simulink model "GFo_29bus"  (R2017a)
settings: Solver=ode1  StartTime=0.0  StopTime=4.5  FixedStep=Time_Step  RelTol=1e-3  EnableMultiTasking=on
PreLoadFcn:
  | Init_29bus;
InitFcn:
  | Init_29bus;
values from neighbouring files (symbols this model uses):
  Time_Step = 40e-6    (= 4e-05)    [Init_29bus.m]
  VSC01_Delta_P_Time_Step = 2    [Init_29bus.m]
  VSC01_Delta_P_Value = -0.2    [Init_29bus.m]
undefined symbols (not defined in the file or in its folder): D1, D11, Delta
libraries: powerlib x168, sps_avr x6, GFo_Lib x1
(part 2 of 5)

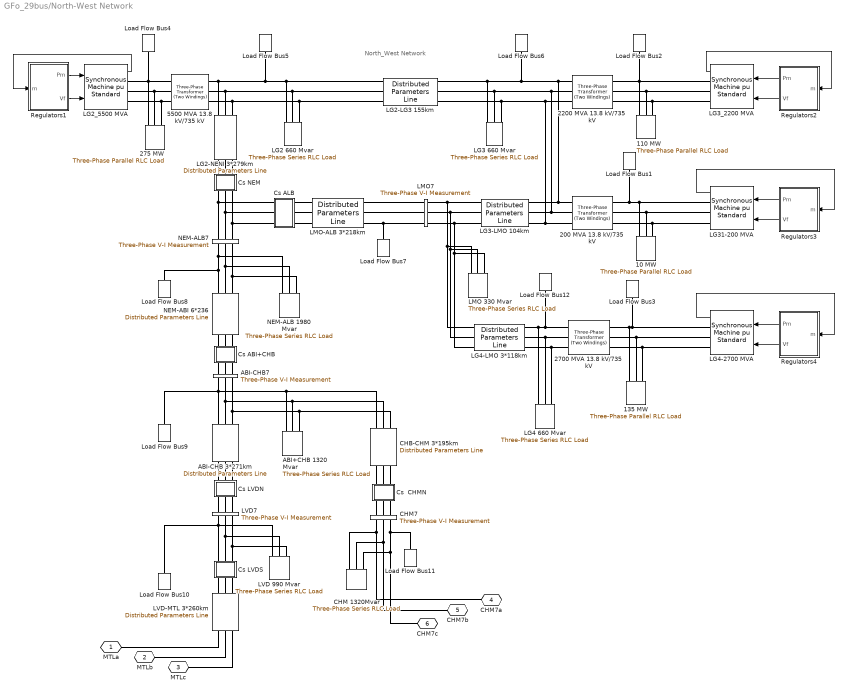
== system GFo_29bus/North-West Network ==
  note: North_West Network
  10 MW : powerlib/Elements/Three-Phase Parallel RLC Load  LConnTagsString=A|B|C  Configuration=Y (grounded)  NominalVoltage=(13800)*1  Vabc=[1e3 1e3 1e3]  Vabcp=[1e3 1e3 1e3]  NominalFrequency=60  UnbalancedPower=off  ActivePower=10000000  InductivePower=0  CapacitivePower=0  Pabc=[10e3 9e3 11e3]  QLabc=[100 90 110]  QCabc=[100 90 110]  Pabcp=[10e3 9e3 11e3]  QLabcp=[100 90 110]  QCabcp=[100 90 110]  Measurements=None  LoadType=constant PQ
  110 MW : powerlib/Elements/Three-Phase Parallel RLC Load  LConnTagsString=A|B|C  Configuration=Y (grounded)  NominalVoltage=(13800)*1  Vabc=[1e3 1e3 1e3]  Vabcp=[1e3 1e3 1e3]  NominalFrequency=60  UnbalancedPower=off  ActivePower=110000000  InductivePower=0  CapacitivePower=0  Pabc=[10e3 9e3 11e3]  QLabc=[100 90 110]  QCabc=[100 90 110]  Pabcp=[10e3 9e3 11e3]  QLabcp=[100 90 110]  QCabcp=[100 90 110]  Measurements=None  LoadType=constant PQ
  135 MW : powerlib/Elements/Three-Phase Parallel RLC Load  LConnTagsString=A|B|C  Configuration=Y (grounded)  NominalVoltage=(13800)*1  Vabc=[1e3 1e3 1e3]  Vabcp=[1e3 1e3 1e3]  NominalFrequency=60  UnbalancedPower=off  ActivePower=135000000  InductivePower=0  CapacitivePower=0  Pabc=[10e3 9e3 11e3]  QLabc=[100 90 110]  QCabc=[100 90 110]  Pabcp=[10e3 9e3 11e3]  QLabcp=[100 90 110]  QCabcp=[100 90 110]  Measurements=None  LoadType=constant PQ
  200 MVA 13.8 kV/735 kV : powerlib/Elements/Three-Phase Transformer (Two Windings)  Winding1Connection=Delta (D1)  Winding2Connection=Yg  CoreType=Three single-phase transformers  SetSaturation=off  Hysteresis=off  DataFile='basic_model'  SetInitialFlux=off  Measurements=None  UNITS=pu  NominalPower=[ 200e6 60 ]  Winding1="[ 13.8e3 0.002  0.0]"  Winding2=[ 735e3 0.002 0.12]  Rm=500  Lm=500  L0=0.5  Saturation="[ 0,0  ;  0.005,1.2  ;  1.0,1.4 ]"  InitialFluxes=[ 0.8 , -0.8 , 0.7 ]  MoreParameters=off  BreakLoop=off  DataType=off  TransfoNumber=0
  2200 MVA 13.8 kV/735 kV : powerlib/Elements/Three-Phase Transformer (Two Windings)  Winding1Connection=Delta (D1)  Winding2Connection=Yg  CoreType=Three single-phase transformers  SetSaturation=off  Hysteresis=off  DataFile='basic_model'  SetInitialFlux=off  Measurements=None  UNITS=pu  NominalPower=[ 2200e6 60 ]  Winding1="[ 13.8e3 0.002  0.0]"  Winding2=[ 735e3 0.002 0.12]  Rm=500  Lm=500  L0=0.5  Saturation="[ 0,0  ;  0.005,1.2  ;  1.0,1.4 ]"  InitialFluxes=[ 0.8 , -0.8 , 0.7 ]  MoreParameters=off  BreakLoop=off  DataType=off  TransfoNumber=0
  2700 MVA 13.8 kV/735 kV : powerlib/Elements/Three-Phase Transformer (Two Windings)  Winding1Connection=Delta (D1)  Winding2Connection=Yg  CoreType=Three single-phase transformers  SetSaturation=off  Hysteresis=off  DataFile='basic_model'  SetInitialFlux=off  Measurements=None  UNITS=pu  NominalPower=[ 2700e6 60 ]  Winding1="[ 13.8e3 0.002  0.0]"  Winding2=[ 735e3 0.002 0.12]  Rm=500  Lm=500  L0=0.5  Saturation="[ 0,0  ;  0.005,1.2  ;  1.0,1.4 ]"  InitialFluxes=[ 0.8 , -0.8 , 0.7 ]  MoreParameters=off  BreakLoop=off  DataType=off  TransfoNumber=0
  275 MW : powerlib/Elements/Three-Phase Parallel RLC Load  LConnTagsString=A|B|C  Configuration=Y (grounded)  NominalVoltage=(13800)*1  Vabc=[1e3 1e3 1e3]  Vabcp=[1e3 1e3 1e3]  NominalFrequency=60  UnbalancedPower=off  ActivePower=275000000  InductivePower=0  CapacitivePower=0  Pabc=[10e3 9e3 11e3]  QLabc=[100 90 110]  QCabc=[100 90 110]  Pabcp=[10e3 9e3 11e3]  QLabcp=[100 90 110]  QCabcp=[100 90 110]  Measurements=None  LoadType=constant PQ
  5500 MVA 13.8 kV/735 kV : powerlib/Elements/Three-Phase Transformer (Two Windings)  Winding1Connection=Delta (D1)  Winding2Connection=Yg  CoreType=Three single-phase transformers  SetSaturation=off  Hysteresis=off  DataFile='basic_model'  SetInitialFlux=off  Measurements=None  UNITS=pu  NominalPower=[ 5500e6 60 ]  Winding1="[ 13.8e3 0.002  0.0]"  Winding2=[ 735e3 0.002 0.12]  Rm=500  Lm=500  L0=0.5  Saturation="[ 0,0  ;  0.005,1.2  ;  1.0,1.4 ]"  InitialFluxes=[ 0.8 , -0.8 , 0.7 ]  MoreParameters=off  BreakLoop=off  DataType=off  TransfoNumber=0
  ABI+CHB 1320 Mvar : powerlib/Elements/Three-Phase Series RLC Load  LConnTagsString=A|B|C  Configuration=Y (grounded)  NominalVoltage=735e3  Vabc=[1e3 1e3 1e3]  Vabcp=[1e3 1e3 1e3]  NominalFrequency=60  UnbalancedPower=off  ActivePower=4400000  InductivePower=1320e6  CapacitivePower=0  Pabc=[10e3 9e3 11e3]  QLabc=[100 90 110]  QCabc=[100 90 110]  Pabcp=[10e3 9e3 11e3]  QLabcp=[100 90 110]  QCabcp=[100 90 110]  Measurements=None  LoadType=constant Z
  ABI-CHB 3*271km : powerlib/Elements/Distributed Parameters Line  Phases=3  Frequency=60  Resistance="[0.01273  0.3864]/3"  Inductance="[0.9337e-3  4.1264e-3]/3"  Capacitance=[12.74e-9 7.751e-9]*3  Length=271  x1=[-0.00156 9.5951452421556e-08 0 0;-0.00152 9.70899498769542e-08 0 0;-0.00148 9.82063699150184e-08 0 0;-0.00144 9.93004586714597e-08 0 0;-0.0014 1.0037196735993e-07 0 0;-0.00136 1.01420652328593e-07 0 0;-0.00132 1.02446275115531e-07 0 0;-0.00128 1.03448602502967e-07 0 0;-0.00124 1.04427406570297e-07 0 0;-0.0012 1.05382464745916e-07 0 0;-0.00116 1.06313559857832e-07 0 0;-0.00112 1.07220480183045e-07 0 0;-0.00108 1.08103019495694e-07 0 0;-0.00104 1.08960977113951e-07 0 0;-0.001 1.09794157945652e-07 0 0;-0.00096 1.1060237253266e-07 216619.58458071 -655246.59132654;-0.00092 1.11385437093949e-07 226475.422537365 -651905.728699672;-0.00088 1.12143173567389e-07 236279.761935975 -648416.628331894;-0.00084 1.12875409650242e-07 246030.373354311 -644780.083614539;-0.0008 1.13581978838336e-07 255725.039587421 -640996.921466518;-0.00076 1.14262720463932e-07 265361.556151809 -637068.002146277;-0.00072 1.14917479732254e-07 274937.731786708 -632994.219056188;-0.00068 1.15546107756691e-07 284451.38895236 -628776.498539396;-0.00064 1.16148461592652e-07 293900.36432517 -624415.799669173;-0.0006 1.16724404270068e-07 303282.50928962 -619913.114030838;-0.00056 1.17273804824541e-07 312595.690426855 -615269.465496275;-0.00052 1.17796538327124e-07 321837.789999797 -610485.909991117;-0.00048 1.18292485912725e-07 331006.706434705 -605563.535254633;-0.00044 1.1876153480714e-07 340100.354799049 -600503.460592389;-0.0004 1.19203578352696e-07 349116.667275612 -595306.836621728;-0.00036 1.19618516032503e-07 358053.593632691 -589974.845010127;-0.00032 1.20006253493309e-07 366909.101690301 -584508.698206496;-0.00028 1.20366702566962e-07 375681.177782275 -578909.639165482;-0.00024 1.20699781290449e-07 384367.827214159 -573178.941064826;-0.0002 1.21005413924541e-07 392967.074716781 -567317.907015856;-0.00016 1.21283530971012e-07 401476.964895416 -561327.869767173;-0.00012 1.21534069188446e-07 409895.562674423 -555210.191401589;-8e-05 1.21756971606611e-07 418220.953737267 -548966.26302641;-4e-05 1.21952187539421e-07 426451.244961816 -542597.504457102]  x2=[-0.00156 2.08994673487687e-07 0 0;-0.00152 2.11355075811643e-07 0 0;-0.00148 2.13667417814008e-07 0 0;-0.00144 2.15931173688151e-07 0 0;-0.0014 2.18145828675509e-07 0 0;-0.00136 2.20310879182635e-07 0 0;-0.00132 2.22425832895715e-07 0 0;-0.00128 2.24490208892514e-07 0 0;-0.00124 2.26503537751732e-07 0 0;-0.0012 2.28465361659748e-07 0 0;-0.00116 2.30375234514724e-07 0 0;-0.00112 2.32232722028042e-07 0 0;-0.00108 2.34037401823062e-07 0 0;-0.00104 2.35788863531159e-07 0 0;-0.001 2.37486708885046e-07 0 0;-0.00096 2.39130551809331e-07 -50306.9183180223 -677474.462196763;-0.00092 2.40720018508308e-07 -40085.5444534979 -678156.068059365;-0.00088 2.42254747550957e-07 -29855.0554818478 -678683.467080259;-0.00084 2.4373438995313e-07 -19617.7777280401 -679056.539333457;-0.0008 2.45158609256902e-07 -9376.03906075358 -679275.199985543;-0.00076 2.46527081607088e-07 867.831636959905 -679339.399314973;-0.00072 2.47839495824875e-07 11111.5049972429 -679249.122723373;-0.00068 2.49095553478589e-07 21352.6516971111 -679004.390738859;-0.00064 2.5029496895155e-07 31588.9429881209 -678605.259011377;-0.0006 2.51437469507023e-07 41818.0512259065 -678051.818300037;-0.00056 2.52522795350234e-07 52037.6503994669 -677344.194452486;-0.00052 2.53550699687447e-07 62245.4166600801 -676482.548376285;-0.00048 2.5452094878208e-07 72439.0288497263 -675467.076002319;-0.00044 2.55433322007854e-07 82616.1690288997 -674298.00824025;-0.0004 2.56287611898967e-07 92774.5230036874 -672975.610926006;-0.00036 2.57083624197264e-07 102911.780851998 -671500.184761332;-0.00032 2.57821177896413e-07 113025.637448815 -669872.065245414;-0.00028 2.58500105283064e-07 123113.792990369 -668091.62259859;-0.00024 2.59120251974984e-07 133173.953517084 -666159.261678164;-0.0002 2.59681476956162e-07 143203.831435213 -664075.421886345;-0.00016 2.60183652608878e-07 153201.146037011 -661840.577070332;-0.00012 2.6062666474272e-07 163163.624019351 -659455.235414563;-8e-05 2.61010412620547e-07 173089.000000652 -656919.93932516;-4e-05 2.61334808981402e-07 182975.017036008 -654235.265306591]  x3=[-0.00156 -1.04791549679137e-10 0 0;-0.00152 -8.57007981393384e-11 0 0;-0.00148 -6.65905589770951e-11 0 0;-0.00144 -4.74651776959928e-11 0 0;-0.0014 -2.83290032428046e-11 0 0;-0.00136 -9.18638701857813e-12 0 0;-0.00132 9.95831811083642e-12 0 0;-0.00128 2.91007588045895e-11 0 0;-0.00124 4.82365822367446e-11 0 0;-0.0012 6.73614370860738e-11 0 0;-0.00116 8.64709745255098e-11 0 0;-0.00112 1.05560849211033e-10 0 0;-0.00108 1.24626720269763e-10 0 0;-0.00104 1.43664252287039e-10 0 0;-0.001 1.62669116292252e-10 0 0;-0.00096 1.8163699074322e-10 85.0496761443598 864.700572722881;-0.00092 2.00563562508863e-10 72.0004876131748 865.884385233979;-0.00088 2.19444527849978e-10 58.9349267920121 866.871303102944;-0.00084 2.38275593397869e-10 45.8559646767302 867.661101913164;-0.0008 2.57052477130623e-10 32.7665753105259 868.253602071198;-0.00076 2.75770909346803e-10 19.6697351076627 868.648668847622;-0.00072 2.94426633636345e-10 6.56842217666069 868.846212407657;-0.00068 3.13015407848425e-10 -6.53438435690062 868.846187831601;-0.00064 3.3153300505609e-10 -19.6357050278094 868.648595125043;-0.0006 3.49975214517425e-10 -32.7325607087259 868.25347921886;-0.00056 3.68337842633035e-10 -45.8219732876108 867.660929959001;-0.00052 3.86616713899642e-10 -58.9009663449219 866.871082086059;-0.00048 4.04807671859548e-10 -71.9665658304266 865.884115204629;-0.00044 4.22906580045786e-10 -85.0158007394746 864.700253742467;-0.0004 4.40909322922712e-10 -98.0457037885795 863.319766899462;-0.00036 4.58811806821846e-10 -111.053312090153 861.742968586416;-0.00032 4.76609960872733e-10 -124.03566782624 859.970217353669;-0.00028 4.94299737928627e-10 -136.989818921102 858.001916309563;-0.00024 5.11877115486776e-10 -149.912819712491 855.838513028782;-0.0002 5.29338096603103e-10 -162.80173162147 853.480499450574;-0.00016 5.46678710801079e-10 -175.653623820621 850.928411766894;-0.00012 5.63895014974577e-10 -188.465573900487 848.182830300473;-8e-05 5.80983094284492e-10 -201.234668534106 845.244379372858;-4e-05 5.97939063048952e-10 -213.958004139475 842.113727162451]  x4=[-0.00156 9.60954535339062e-10 0 0;-0.00152 9.59976323627074e-10 0 0;-0.00148 9.58779821577575e-10 0 0;-0.00144 9.57365301264816e-10 0 0;-0.0014 9.55733084338515e-10 0 0;-0.00136 9.53883541950726e-10 0 0;-0.00132 9.5181709467144e-10 0 0;-0.00128 9.49534212392946e-10 0 0;-0.00124 9.47035414222988e-10 0 0;-0.0012 9.44321268366722e-10 0 0;-0.00116 9.41392391997508e-10 0 0;-0.00112 9.38249451116577e-10 0 0;-0.00108 9.34893160401581e-10 0 0;-0.00104 9.31324283044084e-10 0 0;-0.001 9.27543630576022e-10 0 0;-0.00096 9.23552062685162e-10 -872.254416614129 -15817.4970067936;-0.00092 9.19350487019622e-10 -633.642051346427 -15828.8524142298;-0.00088 9.14939858981474e-10 -394.885601340545 -15836.6084771291;-0.00084 9.10321181509499e-10 -156.039357754267 -15840.7634318299;-0.0008 9.05495504851124e-10 82.8423678363377 -15841.3163335312;-0.00076 9.00463926323607e-10 321.7052557869 -15838.2670565079;-0.00072 8.95227590064514e-10 560.494990736563 -15831.6162941394;-0.00068 8.89787686771555e-10 799.157273958836 -15821.3655587517;-0.00064 8.84145453431825e-10 1037.63783570865 -15807.5171812735;-0.0006 8.78302173040531e-10 1275.88244756283 -15790.0743107065;-0.00056 8.72259174309243e-10 1513.83693475118 -15769.0409134091;-0.00052 8.6601783136376e-10 1751.44718847534 -15744.4217721944;-0.00048 8.59579563431644e-10 1988.65917821267 -15716.2224852428;-0.00044 8.52945834519503e-10 2225.41896400235 -15684.449464829;-0.0004 8.46118153080083e-10 2461.67270871081 -15649.1099358638;-0.00036 8.39098071669265e-10 2697.36669027387 -15610.2119342514;-0.00032 8.31887186593023e-10 2932.44731391266 -15567.7643050618;-0.00028 8.24487137544439e-10 3166.86112432061 -15521.77670052;-0.00024 8.16899607230852e-10 3400.55481781874 -15472.2595778106;-0.0002 8.09126320991223e-10 3633.47525447644 -15419.2241967002;-0.00016 8.01169046403809e-10 3865.56947019502 -15362.6826169773;-0.00012 7.9302959288423e-10 4096.78468875133 -15302.6476957094;-8e-05 7.84709811274025e-10 4327.06833379859 -15239.1330843199;-4e-05 7.76211593419786e-10 4556.36804082179 -15172.1532254837]  x5=0.00153261764655846  V1=ones(3,3)  V2=ones(3,3)  I1=ones(3,3)  I2=ones(3,3)  nHarmo=1  Measurements=None
      settings: AttributesFormatString=\n  SourceProductName=Simscape Power Systems
  ABI-CHB7 : powerlib/Measurements/Three-Phase V-I Measurement  VoltageMeasurement=no  SetLabelV=on  LabelV=Vabc_ABI7  Vpu=on  VpuLL=off  CurrentMeasurement=no  SetLabelI=off  LabelI=A1  Ipu=off  Pbase=100e6  Vbase=500e3  OutputType=Magnitude  PhasorSimulation=off  PSBequivalent=0
  CHB-CHM 3*195km : powerlib/Elements/Distributed Parameters Line  Phases=3  Frequency=60  Resistance="[0.01273  0.3864]/3"  Inductance="[0.9337e-3  4.1264e-3]/3"  Capacitance=[12.74e-9 7.751e-9]*3  Length=195  x1=[-0.00112 1.07244333430672e-07 0 0;-0.00108 1.08126069397218e-07 0 0;-0.00104 1.08983218428023e-07 0 0;-0.001 1.09815585614788e-07 0 0;-0.00096 1.10622981684394e-07 0 0;-0.00092 1.11405223041937e-07 0 0;-0.00088 1.12162131812478e-07 0 0;-0.00084 1.12893535881489e-07 0 0;-0.0008 1.13599268933994e-07 0 0;-0.00076 1.14279170492381e-07 0 0;-0.00072 1.149330859529e-07 0 0;-0.00068 1.15560866620814e-07 284451.38895236 -628776.498539396;-0.00064 1.16162369744213e-07 293900.36432517 -624415.799669173;-0.0006 1.16737458546474e-07 303282.50928962 -619913.114030838;-0.00056 1.17286002257362e-07 312595.690426855 -615269.465496275;-0.00052 1.17807876142768e-07 321837.789999797 -610485.909991117;-0.00048 1.18302961533072e-07 331006.706434705 -605563.535254633;-0.00044 1.18771145850124e-07 340100.354799049 -600503.460592389;-0.0004 1.19212322632848e-07 349116.667275612 -595306.836621728;-0.00036 1.19626391561449e-07 358053.593632691 -589974.845010127;-0.00032 1.20013258480223e-07 366909.101690301 -584508.698206496;-0.00028 1.20372835418969e-07 375681.177782275 -578909.639165482;-0.00024 1.20705040612991e-07 384367.827214159 -573178.941064826;-0.0002 1.21009798521694e-07 392967.074716781 -567317.907015856;-0.00016 1.21287039845758e-07 401476.964895416 -561327.869767173;-0.00012 1.21536701542895e-07 409895.562674423 -555210.191401589;-8e-05 1.2175872684219e-07 418220.953737267 -548966.26302641;-4e-05 1.21953065257003e-07 426451.244961816 -542597.504457102]  x2=[-0.00112 7.55642474220007e-08 0 0;-0.00108 7.61098867769976e-08 0 0;-0.00104 7.6638219400085e-08 0 0;-0.001 7.71491251529807e-08 0 0;-0.00096 7.76424878601224e-08 0 0;-0.00092 7.8118195335085e-08 0 0;-0.00088 7.8576139406091e-08 0 0;-0.00084 7.90162159406078e-08 0 0;-0.0008 7.94383248690265e-08 0 0;-0.00076 7.9842370207417e-08 0 0;-0.00072 8.02282600793536e-08 0 0;-0.00068 8.05959067368072e-08 200726.403510761 -641022.029740575;-0.00064 8.09452265800983e-08 210369.549035787 -637922.423631795;-0.0006 8.1276140176907e-08 219964.858339513 -634677.75946509;-0.00056 8.15885722803351e-08 229510.149531348 -631288.775049111;-0.00052 8.18824518460165e-08 239003.25209439 -627756.241009687;-0.00048 8.21577120482723e-08 248442.007378983 -624080.960614598;-0.00044 8.24142902953063e-08 257824.26909357 -620263.76959091;-0.0004 8.26521282434376e-08 267147.903792748 -616305.535934943;-0.00036 8.28711718103681e-08 276410.791362388 -612207.159714898;-0.00032 8.30713711874794e-08 285610.825501738 -607969.572866183;-0.00028 8.32526808511596e-08 294745.914202371 -603593.738979505;-0.00024 8.34150595731549e-08 303813.980223895 -599080.653081753;-0.0002 8.3558470429944e-08 312812.961566297 -594431.341409743;-0.00016 8.3682880811135e-08 321740.811938822 -589646.861176853;-0.00012 8.37882624268799e-08 330595.501225287 -584728.300332629;-8e-05 8.38745913143081e-08 339375.015945708 -579676.777315392;-4e-05 8.39418478429752e-08 348077.359714148 -574493.440797913]  x3=[-0.00112 4.95882150276911e-10 0 0;-0.00108 4.95457745542146e-10 0 0;-0.00104 4.9492067798869e-10 0 0;-0.001 4.94271069741073e-10 0 0;-0.00096 4.9350906851461e-10 0 0;-0.00092 4.92634847581807e-10 0 0;-0.00088 4.91648605732966e-10 0 0;-0.00084 4.90550567230979e-10 0 0;-0.0008 4.89340981760331e-10 0 0;-0.00076 4.88020124370327e-10 0 0;-0.00072 4.86588295412549e-10 0 0;-0.00068 4.85045820472552e-10 1577.42073477442 -3661.80221392756;-0.00064 4.83393050295836e-10 1632.45704438713 -3637.60049775401;-0.0006 4.81630360708088e-10 1687.12214734566 -3612.57162259661;-0.00056 4.79758152529718e-10 1741.403613277 -3586.72127980571;-0.00052 4.7777685148472e-10 1795.28909904391 -3560.05534752636;-0.00048 4.75686908103867e-10 1848.76635155161 -3532.57988936159;-0.00044 4.73488797622261e-10 1901.82321053405 -3504.30115299364;-0.0004 4.71183019871269e-10 1954.44761131904 -3475.22556876332;-0.00036 4.68770099164867e-10 2006.62758757165 -3445.35974820772;-0.00032 4.66250584180416e-10 2058.35127401527 -3414.7104825569;-0.00028 4.63625047833897e-10 2109.60690912964 -3383.28474118956;-0.00024 4.60894087149632e-10 2160.38283782535 -3351.08967004827;-0.0002 4.58058323124531e-10 2210.66751409409 -3318.13259001459;-0.00016 4.55118400586877e-10 2260.44950363411 -3284.42099524429;-0.00012 4.52074988049705e-10 2309.71748645029 -3249.96255146331;-8e-05 4.48928777558778e-10 2358.4602594282 -3214.76509422461;-4e-05 4.45680484535232e-10 2406.66673888162 -3178.83662712644]  x4=[-0.00112 1.21600407393123e-10 0 0;-0.00108 1.29687420233768e-10 0 0;-0.00104 1.3774494327343e-10 0 0;-0.001 1.45771144300853e-10 0 0;-0.00096 1.53764198227138e-10 0 0;-0.00092 1.61722287500753e-10 0 0;-0.00088 1.69643602520824e-10 0 0;-0.00084 1.77526342048625e-10 0 0;-0.0008 1.85368713617167e-10 0 0;-0.00076 1.93168933938784e-10 0 0;-0.00072 2.00925229310641e-10 0 0;-0.00068 2.08635836018058e-10 1976.82314553332 -10994.7955965049;-0.00064 2.16299000735563e-10 2142.38966517679 -10963.7374282637;-0.0006 2.23912980925585e-10 2307.46902388557 -10930.1862006786;-0.00056 2.31476045234687e-10 2472.0236840371 -10894.1495430093;-0.00052 2.38986473887267e-10 2636.01622732069 -10855.6356496811;-0.00048 2.46442559076617e-10 2799.40936324623 -10814.6532784211;-0.00044 2.53842605353263e-10 2962.16593762364 -10771.2117482673;-0.0004 2.61184930010497e-10 3124.24894101147 -10725.3209374489;-0.00036 2.6846786346701e-10 3285.62151713249 -10676.9912811405;-0.00032 2.75689749646538e-10 3446.2469712545 -10626.2337690892;-0.00028 2.82848946354444e-10 3606.08877853442 -10573.0599431156;-0.00024 2.89943825651134e-10 3765.11059232369 -10517.4818944891;-0.0002 2.96972774222241e-10 3923.2762524332 -10459.5122611787;-0.00016 3.03934193745473e-10 4080.54979335579 -10399.1642249791;-0.00012 3.10826501254065e-10 4236.89545244454 -10336.4515085133;-8e-05 3.17648129496725e-10 4392.27767804483 -10271.3883721123;-4e-05 3.24397527294018e-10 4546.66113757852 -10203.9896105721]  x5=0.0011028060556417  V1=ones(3,3)  V2=ones(3,3)  I1=ones(3,3)  I2=ones(3,3)  nHarmo=1  Measurements=None
      settings: AttributesFormatString=\n  SourceProductName=Simscape Power Systems
  CHM 1320Mvar : powerlib/Elements/Three-Phase Series RLC Load  LConnTagsString=A|B|C  Configuration=Y (grounded)  NominalVoltage=735e3  Vabc=[1e3 1e3 1e3]  Vabcp=[1e3 1e3 1e3]  NominalFrequency=60  UnbalancedPower=off  ActivePower=4400000  InductivePower=1320e6  CapacitivePower=0  Pabc=[10e3 9e3 11e3]  QLabc=[100 90 110]  QCabc=[100 90 110]  Pabcp=[10e3 9e3 11e3]  QLabcp=[100 90 110]  QCabcp=[100 90 110]  Measurements=None  LoadType=constant Z
  CHM7 : powerlib/Measurements/Three-Phase V-I Measurement  VoltageMeasurement=no  SetLabelV=on  LabelV=Vabc_CHM7  Vpu=on  VpuLL=off  CurrentMeasurement=no  SetLabelI=off  LabelI=A1  Ipu=off  Pbase=100e6  Vbase=735e3  OutputType=Magnitude  PhasorSimulation=off  PSBequivalent=0
  "Cs  CHMN " : Subsystem  mask{Xc=25/3}
      mask prompts: Xc "Condensator Reactance at  60Hz  (ohm):"
      mask help: Series Compensation
      mask init:
      | Cs=1/Xc/(2*pi*60);
      mask Display: disp('Cs')
  "Cs ABI+CHB " : Subsystem  mask{Xc=25/6}
      mask prompts: Xc "Condensator Reactance at  60Hz  (ohm):"
      mask help: Series Compensation
      mask init:
      | Cs=1/Xc/(2*pi*60);
      mask Display: disp('Cs')
  Cs ALB : Subsystem  mask{Xc=16/3}
      mask prompts: Xc "Reactance @ 60Hz du condensateur (ohm):"
      mask init:
      | Cs=1/Xc/(2*pi*60);
      mask Display: disp('Cs')
  "Cs LVDN " : Subsystem  mask{Xc=34/3}
      mask prompts: Xc "Condensator Reactance at  60Hz  (ohm):"
      mask help: Series Compensation
      mask init:
      | Cs=1/Xc/(2*pi*60);
      mask Display: disp('Cs')
  "Cs LVDS " : Subsystem  mask{Xc=34/3}
      mask prompts: Xc "Condensator Reactance at  60Hz  (ohm):"
      mask help: Series Compensation
      mask init:
      | Cs=1/Xc/(2*pi*60);
      mask Display: disp('Cs')
  "Cs NEM " : Subsystem  mask{Xc=16/3}
      mask prompts: Xc "Condensator Reactance at  60Hz  (ohm):"
      mask help: Series Compensation
      mask init:
      | Cs=1/Xc/(2*pi*60);
      mask Display: disp('Cs')
  LG2 660 Mvar : powerlib/Elements/Three-Phase Series RLC Load  LConnTagsString=A|B|C  Configuration=Y (grounded)  NominalVoltage=735e3  Vabc=[1e3 1e3 1e3]  Vabcp=[1e3 1e3 1e3]  NominalFrequency=60  UnbalancedPower=off  ActivePower=2200000  InductivePower=660e6  CapacitivePower=0  Pabc=[10e3 9e3 11e3]  QLabc=[100 90 110]  QCabc=[100 90 110]  Pabcp=[10e3 9e3 11e3]  QLabcp=[100 90 110]  QCabcp=[100 90 110]  Measurements=None  LoadType=constant Z
  LG2-LG3 155km : powerlib/Elements/Distributed Parameters Line  Phases=3  Frequency=60  Resistance="[0.01273  0.3864]"  Inductance="[0.9337e-3  4.1264e-3]"  Capacitance=[12.74e-9 7.751e-9]  Length=155  x1=[-0.00088 4.73235624331992e-09 492216.116306252 -498778.900482482;-0.00084 4.72947863230192e-09 499681.229064062 -491300.088111067;-0.0008 4.72552557862823e-09 507032.71861945 -483709.558336407;-0.00076 4.72049798118915e-09 514268.913307088 -476009.037179515;-0.00072 4.71439698321699e-09 521388.167678706 -468200.275672495;-0.00068 4.70722397202608e-09 528388.862877254 -460285.049460374;-0.00064 4.69898057869729e-09 535269.407005016 -452265.158397336;-0.0006 4.6896686777072e-09 542028.235485591 -444142.426137446;-0.00056 4.67929038650177e-09 548663.811419669 -435918.699719975;-0.00052 4.66784806501494e-09 555174.625934506 -427595.849149389;-0.00048 4.65534431513192e-09 561559.198527027 -419175.766970137;-0.00044 4.64178198009763e-09 567816.077400483 -410660.367836293;-0.0004 4.62716414387009e-09 573943.839794576 -402051.588076187;-0.00036 4.61149413041919e-09 579941.09230898 -393351.385252099;-0.00032 4.59477550297087e-09 585806.471220193 -384561.737715121;-0.00028 4.57701206319682e-09 591538.642791629 -375684.644155307;-0.00024 4.55820785035008e-09 597136.303576907 -366722.123147178;-0.0002 4.53836714034648e-09 602598.180716236 -357676.212690722;-0.00016 4.51749444479238e-09 607923.032225855 -348548.969747969;-0.00012 4.49559450995874e-09 613109.647280451 -339342.469775253;-8e-05 4.47267231570189e-09 618156.846488488 -330058.806251276;-4e-05 4.44873307433114e-09 623063.48216039 -320700.090201062]  x2=[-0.00088 -1.8594565706245e-09 498841.55452554 -488122.876382841;-0.00084 -1.90046755388394e-09 506145.233646554 -480545.374264078;-0.0008 -1.94104638721055e-09 513333.819706248 -472858.600271255;-0.00076 -1.98118384332758e-09 520405.678082143 -465064.302310489;-0.00072 -2.02087079532365e-09 527359.200694629 -457164.252737921;-0.00068 -2.0600982187281e-09 534192.80637263 -449160.247956698;-0.00064 -2.09885719356314e-09 540904.941213144 -441054.108008481;-0.0006 -2.13713890637215e-09 547494.078934592 -432847.676159593;-0.00056 -2.17493465222374e-09 553958.721223878 -424542.818481865;-0.00052 -2.21223583669126e-09 560297.398077094 -416141.423428316;-0.00048 -2.24903397780702e-09 566508.668133786 -407645.401403729;-0.00044 -2.28532070799107e-09 572591.119004707 -399056.684330248;-0.0004 -2.32108777595389e-09 578543.367592983 -390377.225208069;-0.00036 -2.35632704857267e-09 584364.060408613 -381608.997671347;-0.00032 -2.3910305127407e-09 590051.873876247 -372753.99553941;-0.00028 -2.4251902771895e-09 595605.514636152 -363814.232363381;-0.00024 -2.45879857428322e-09 601023.719838313 -354791.740968313;-0.0002 -2.49184776178493e-09 606305.25742959 -345688.572990943;-0.00016 -2.52433032459438e-09 611448.926433881 -336506.798413165;-0.00012 -2.55623887645692e-09 616453.557225212 -327248.50509134;-8e-05 -2.58756616164302e-09 621318.011793699 -317915.798281528;-4e-05 -2.61830505659818e-09 626041.184004323 -308510.800160775]  x3=[-0.00088 9.57977380688901e-12 1822.65778344413 -2130.15037170099;-0.00084 9.18431506304634e-12 1854.57117293959 -2102.42438377255;-0.0008 8.78676788516048e-12 1886.06284894347 -2074.22032266978;-0.00076 8.3872226720314e-12 1917.1256505202 -2045.54460175295;-0.00072 7.98577027679503e-12 1947.7525142566 -2016.40374163371;-0.00068 7.58250198626407e-12 1977.93647586796 -1986.80436869234;-0.00064 7.17750950017013e-12 2007.6706717817 -1956.75321357101;-0.0006 6.77088491031207e-12 2036.94834069809 -1926.25710964323;-0.00056 6.36272067961503e-12 2065.76282512771 -1895.32299146005;-0.00052 5.95310962110521e-12 2094.10757290527 -1863.95789317318;-0.00048 5.54214487680498e-12 2121.97613867956 -1832.16894693549;-0.00044 5.12991989655318e-12 2149.36218537906 -1799.96338127922;-0.0004 4.71652841675546e-12 2176.25948565292 -1767.34851947228;-0.00036 4.30206443906937e-12 2202.661923287 -1734.33177785297;-0.00032 3.88662220902926e-12 2228.56349459468 -1700.92066414361;-0.00028 3.47029619461563e-12 2253.95830978199 -1667.12277574334;-0.00024 3.05318106477389e-12 2278.84059428697 -1632.94579800053;-0.0002 2.63537166788754e-12 2303.2046900927 -1598.39750246517;-0.00016 2.21696301021039e-12 2327.04505701389 -1563.48574512175;-0.00012 1.79805023426299e-12 2350.35627395669 -1528.21846460281;-8e-05 1.37872859719805e-12 2373.13304015141 -1492.60368038382;-4e-05 9.59093449139748e-13 2395.37017635782 -1456.64949095957]  x4=[-0.00088 -6.8062295315058e-12 1450.90460658014 -1864.19450277471;-0.00084 -6.45732020575493e-12 1478.84974910908 -1842.10455115884;-0.0008 -6.10694254107482e-12 1506.45861395813 -1819.59572085367;-0.00076 -5.7551762103249e-12 1533.72492310951 -1796.6731301731;-0.00072 -5.40210120213528e-12 1560.64247643966 -1773.34199151658;-0.00068 -5.04779780271803e-12 1587.20515312907 -1749.60761018384;-0.00064 -4.6923465776108e-12 1613.40691305413 -1725.47538316852;-0.0006 -4.33582835335689e-12 1639.2417981606 -1700.95079793093;-0.00056 -3.97832419912602e-12 1664.70393381838 -1676.03943115027;-0.00052 -3.61991540827988e-12 1689.7875301574 -1650.74694745651;-0.00048 -3.26068347988671e-12 1714.48688338418 -1625.07909814234;-0.00044 -2.90071010018915e-12 1738.79637707878 -1599.04171985533;-0.0004 -2.54007712402947e-12 1762.71048347197 -1572.64073327078;-0.00036 -2.17886655623648e-12 1786.22376470219 -1545.88214174535;-0.00032 -1.81716053297834e-12 1809.33087405206 -1518.77202995202;-0.00028 -1.45504130308553e-12 1832.02655716417 -1491.3165624964;-0.00024 -1.09259120934814e-12 1854.3056532359 -1463.52198251504;-0.0002 -7.29892669791852e-13 1876.16309619294 -1435.39461025573;-0.00016 -3.67028158936777e-13 1897.59391584125 -1406.94084164037;-0.00012 -4.08018904347539e-15 1918.59323899724 -1378.16714681056;-8e-05 3.58868708649629e-13 1939.15629059594 -1349.08006865637;-4e-05 7.21736002693137e-13 1959.27839477672 -1319.68622132853]  x5=0.000876589428843401  V1=ones(3,3)  V2=ones(3,3)  I1=ones(3,3)  I2=ones(3,3)  nHarmo=1  Measurements=None
      settings: AttributesFormatString=\n  SourceProductName=Simscape Power Systems
  LG2-NENI 3*279km : powerlib/Elements/Distributed Parameters Line  Phases=3  Frequency=60  Resistance="[0.01273  0.3864]/3"  Inductance="[0.9337e-3  4.1264e-3]/3"  Capacitance=[12.74e-9 7.751e-9]*3  Length=279  x1=[-0.0016 4.6006914312274e-09 0 0;-0.00156 4.61704685698524e-09 0 0;-0.00152 4.63235240610353e-09 0 0;-0.00148 4.64660459823237e-09 0 0;-0.00144 4.65980019254618e-09 0 0;-0.0014 4.67193618848062e-09 0 0;-0.00136 4.68300982641485e-09 0 0;-0.00132 4.69301858829912e-09 0 0;-0.00128 4.70196019822727e-09 0 0;-0.00124 4.70983262295433e-09 0 0;-0.0012 4.71663407235879e-09 0 0;-0.00116 4.72236299984972e-09 0 0;-0.00112 4.72701810271841e-09 0 0;-0.00108 4.73059832243461e-09 0 0;-0.00104 4.73310284488722e-09 0 0;-0.001 4.73453110056945e-09 469156.140703849 -520528.156335111;-0.00096 4.73488276470827e-09 476951.836643365 -513394.596336102;-0.00092 4.73415775733829e-09 484639.077848285 -506144.294833213;-0.00088 4.73235624331992e-09 492216.116306252 -498778.900482482;-0.00084 4.72947863230192e-09 499681.229064062 -491300.088111067;-0.0008 4.72552557862823e-09 507032.71861945 -483709.558336407;-0.00076 4.72049798118915e-09 514268.913307088 -476009.037179515;-0.00072 4.71439698321699e-09 521388.167678706 -468200.275672495;-0.00068 4.70722397202608e-09 528388.862877254 -460285.049460374;-0.00064 4.69898057869729e-09 535269.407005016 -452265.158397336;-0.0006 4.6896686777072e-09 542028.235485591 -444142.426137446;-0.00056 4.67929038650177e-09 548663.811419669 -435918.699719975;-0.00052 4.66784806501494e-09 555174.625934506 -427595.849149389;-0.00048 4.65534431513192e-09 561559.198527027 -419175.766970137;-0.00044 4.64178198009763e-09 567816.077400483 -410660.367836293;-0.0004 4.62716414387009e-09 573943.839794576 -402051.588076187;-0.00036 4.61149413041919e-09 579941.09230898 -393351.385252099;-0.00032 4.59477550297087e-09 585806.471220193 -384561.737715121;-0.00028 4.57701206319682e-09 591538.642791629 -375684.644155307;-0.00024 4.55820785035008e-09 597136.303576907 -366722.123147178;-0.0002 4.53836714034648e-09 602598.180716236 -357676.212690722;-0.00016 4.51749444479238e-09 607923.032225855 -348548.969747969;-0.00012 4.49559450995874e-09 613109.647280451 -339342.469775253;-8e-05 4.47267231570189e-09 618156.846488488 -330058.806251276;-4e-05 4.44873307433114e-09 623063.48216039 -320700.090201062]  x2=[-0.0016 5.75368748310283e-08 0 0;-0.00156 5.81983011827248e-08 0 0;-0.00152 5.88464937426131e-08 0 0;-0.00148 5.94813051172949e-08 0 0;-0.00144 6.0102590956138e-08 0 0;-0.0014 6.07102099841003e-08 0 0;-0.00136 6.13040240338548e-08 0 0;-0.00132 6.18838980772074e-08 0 0;-0.00128 6.24497002558012e-08 0 0;-0.00124 6.30013019111002e-08 0 0;-0.0012 6.35385776136446e-08 0 0;-0.00116 6.40614051915731e-08 0 0;-0.00112 6.4569665758403e-08 0 0;-0.00108 6.50632437400645e-08 0 0;-0.00104 6.55420269011811e-08 0 0;-0.001 6.60059063705907e-08 282256.24346152 -628817.283710635;-0.00096 6.64547766661023e-08 291706.090402666 -624489.689782335;-0.00092 6.68885357184817e-08 301089.60589442 -620020.092283949;-0.00088 6.73070848946608e-08 310404.65620628 -615409.507563403;-0.00084 6.77103290201665e-08 319649.123176135 -610658.984027902;-0.0008 6.80981764007619e-08 328820.904691916 -605769.601905532;-0.00076 6.84705388432976e-08 337917.915169601 -600742.472999624;-0.00072 6.8827331675765e-08 346938.086027456 -595578.740435938;-0.00068 6.9168473766551e-08 355879.366156415 -590279.578402729;-0.00064 6.9493887542886e-08 364739.722386483 -584846.191883746;-0.0006 6.98034990084834e-08 373517.139949062 -579279.816384227;-0.00056 7.00972377603662e-08 382209.622935091 -573581.717649958;-0.00052 7.0375037004875e-08 390815.1947489 -567753.191379454;-0.00048 7.06368335728574e-08 399331.89855767 -561795.562929326;-0.00044 7.08825679340314e-08 407757.797736399 -555710.187012905;-0.0004 7.11121842105225e-08 416090.976308277 -549498.447392199;-0.00036 7.13256301895694e-08 424329.539380358 -543161.756563228;-0.00032 7.15228573353973e-08 432471.613574446 -536701.555434843;-0.00028 7.1703820800254e-08 440515.347453083 -530119.313001069;-0.00024 7.18684794346081e-08 448458.911940553 -523416.526007072;-0.0002 7.20167957965061e-08 456300.500738791 -516594.718608813;-0.00016 7.21487361600864e-08 464038.33073813 -509655.442026466;-0.00012 7.22642705232481e-08 471670.642422755 -502600.274191683;-8e-05 7.23633726144734e-08 479195.700270808 -495430.81938879;-4e-05 7.24460198988013e-08 486611.793149026 -488148.707889981]  x3=[-0.0016 -1.84837817112506e-10 0 0;-0.00156 -1.78569623872426e-10 0 0;-0.00152 -1.72260825439796e-10 0 0;-0.00148 -1.65912856380975e-10 0 0;-0.00144 -1.59527160169384e-10 0 0;-0.0014 -1.53105188857275e-10 0 0;-0.00136 -1.46648402745542e-10 0 0;-0.00132 -1.40158270051667e-10 0 0;-0.00128 -1.33636266575856e-10 0 0;-0.00124 -1.27083875365455e-10 0 0;-0.0012 -1.20502586377721e-10 0 0;-0.00116 -1.13893896141015e-10 0 0;-0.00112 -1.07259307414506e-10 0 0;-0.00108 -1.00600328846455e-10 0 0;-0.00104 -9.39184746311647e-11 0 0;-0.001 -8.72152641646617e-11 537.641732379249 -985.403191527714;-0.00096 -8.04922216992002e-11 552.439227716164 -977.184734818372;-0.00092 -7.37508759966596e-11 567.11110313673 -968.744074727214;-0.00088 -6.69927599809179e-11 581.654022383001 -960.083130587556;-0.00084 -6.02194103892775e-11 596.064678520552 -951.203871823407;-0.0008 -5.34323674230246e-11 610.339794690451 -942.108317501639;-0.00076 -4.66331743972008e-11 624.476124854383 -932.798535872866;-0.00072 -3.98233773896665e-11 638.470454532777 -923.276643901148;-0.00068 -3.30045248895359e-11 652.319601535744 -913.544806782606;-0.00064 -2.61781674450644e-11 666.020416686686 -903.605237453076;-0.0006 -1.93458573110667e-11 679.56978453839 -893.460196084909;-0.00056 -1.25091480959481e-11 692.96462408145 -883.111989573025;-0.00052 -5.6695944084268e-12 706.201889444866 -872.562971010345;-0.00048 1.17124849597052e-12 719.278570588647 -861.81553915272;-0.00044 8.01182506856025e-12 732.191693988272 -850.872137873473;-0.0004 1.48505798212204e-11 744.938323310835 -839.735255607682;-0.00036 2.16859576800952e-11 757.515560082752 -828.407424786334;-0.00032 2.85164043392053e-11 769.920544348843 -816.891221260471;-0.00028 3.53403666138836e-11 782.15045532266 -805.189263715463;-0.00024 4.21562927939563e-11 794.202512027916 -793.304213075543;-0.0002 4.8962632996588e-11 806.073973930846 -781.238771898734;-0.00016 5.57578395187121e-11 817.762141563391 -768.995683762311;-0.00012 6.25403671889647e-11 829.264357137025 -756.577732638937;-8e-05 6.93086737190437e-11 840.578005147117 -743.987742263609;-4e-05 7.60612200544116e-11 851.700512967675 -731.228575491568]  x4=[-0.0016 3.57962366900935e-10 0 0;-0.00156 3.55285452732805e-10 0 0;-0.00152 3.52527749716575e-10 0 0;-0.00148 3.49689884930128e-10 0 0;-0.00144 3.46772503679446e-10 0 0;-0.0014 3.43776269351866e-10 0 0;-0.00136 3.40701863265235e-10 0 0;-0.00132 3.37549984512986e-10 0 0;-0.00128 3.34321349805165e-10 0 0;-0.00124 3.31016693305464e-10 0 0;-0.0012 3.27636766464271e-10 0 0;-0.00116 3.24182337847803e-10 0 0;-0.00112 3.20654192963338e-10 0 0;-0.00108 3.17053134080597e-10 0 0;-0.00104 3.13379980049316e-10 0 0;-0.001 3.09635566113046e-10 5386.23580507862 -13142.2626920686;-0.00096 3.05820743719225e-10 5583.79617472023 -13059.5498514473;-0.00092 3.01936380325568e-10 5780.08683726433 -12973.8673818105;-0.00088 2.97983359202813e-10 5975.06315790697 -12885.2347666129;-0.00084 2.93962579233875e-10 6168.68080071425 -12793.6721601469;-0.0008 2.89874954709444e-10 6360.8957387039 -12699.2003829597;-0.00076 2.85721415120088e-10 6551.66426385658 -12601.8409171186;-0.00072 2.81502904944889e-10 6740.94299705482 -12501.6159013266;-0.00068 2.77220383436684e-10 6928.68889794694 -12398.548125888;-0.00064 2.72874824403932e-10 7114.85927473413 -12292.6610275261;-0.0006 2.68467215989283e-10 7299.41179387819 -12183.9786840539;-0.00056 2.63998560444881e-10 7482.30448972776 -12072.5258088992;-0.00052 2.5946987390446e-10 7663.49577406101 -11958.3277454845;-0.00048 2.54882186152286e-10 7842.94444554242 -11841.4104614647;-0.00044 2.50236540388992e-10 8020.60969909158 -11721.8005428219;-0.0004 2.45533992994361e-10 8196.45113516196 -11599.5251878203;-0.00036 2.40775613287118e-10 8370.42876892739 -11474.6122008209;-0.00032 2.35962483281774e-10 8542.50303937427 -11347.0899859599;-0.00028 2.31095697442585e-10 8712.6348182974 -11216.9875406893;-0.00024 2.26176362434683e-10 8880.78541919741 -11084.3344491831;-0.0002 2.21205596872425e-10 9046.91660607774 -10949.1608756104;-0.00016 2.16184531065034e-10 9210.99060213912 -10811.4975572761;-0.00012 2.11114306759574e-10 9372.97009836978 -10671.3757976316;-8e-05 2.0599607688133e-10 9532.81826202912 -10528.8274591568;-4e-05 2.00831005271637e-10 9690.4987450232 -10383.8849561145]  x5=0.00157786097191812  V1=ones(3,3)  V2=ones(3,3)  I1=ones(3,3)  I2=ones(3,3)  nHarmo=1  Measurements=None
      settings: AttributesFormatString=\n  SourceProductName=Simscape Power Systems
  LG2_5500 MVA : powerlib/Machines/Synchronous Machine pu Standard  PresetModel=No  MechanicalLoad=Mechanical power Pm  ShowDetailedParameters=on  RotorType=Salient-pole  Units=per unit standard parameters  MeasurementBus=off  NominalParameters="[5500E6  13800   60 ]"  Reactances1=[ 31 32 33 34 35 36 37 ]  Reactances2=[ 1.305, 0.296, 0.252, 0.474, 0.243, 0.18 ]  dAxisTimeConstants=Short-circuit  qAxisTimeConstants=Open-circuit  TimeConstants1=[]  TimeConstants2=[]  TimeConstants3=[]  TimeConstants4=[]  TimeConstants5=[ 1.01, 0.053, 0.1 ]  TimeConstants6=[]  TimeConstants7=[]  TimeConstants8=[]  StatorResistance=2.8544e-3  Mechanical="[ 4.1  0  32]"  PolePairs=32  InitialConditions=[0 -66.6463 0.909698 0.909698 0.909698 0.522896 -119.477 120.523 1.3811]  SetSaturation=off  Saturation=[0.6404,0.7127,0.8441,0.9214,0.9956,1.082,1.19,1.316,1.457;0.7,0.7698,0.8872,0.9466,0.9969,1.046,1.1,1.151,1.201]  LoadFlowParameters=[2 4000000000 0 0 0]  TsPowergui=0  TsBlock=-1  IterativeModel=Trapezoidal non iterative  IterativeDiscreteModel=Trapezoidal non iterative  BusType=swing  Pref=0  Qref=0  Qmin=-Inf  Qmax=Inf  PLF=0  QLF=0
      settings: AttributesFormatString=\n\n  SourceProductName=Simscape Power Systems
  LG3 660 Mvar : powerlib/Elements/Three-Phase Series RLC Load  LConnTagsString=A|B|C  Configuration=Y (grounded)  NominalVoltage=735e3  Vabc=[1e3 1e3 1e3]  Vabcp=[1e3 1e3 1e3]  NominalFrequency=60  UnbalancedPower=off  ActivePower=2200000  InductivePower=660e6  CapacitivePower=0  Pabc=[10e3 9e3 11e3]  QLabc=[100 90 110]  QCabc=[100 90 110]  Pabcp=[10e3 9e3 11e3]  QLabcp=[100 90 110]  QCabcp=[100 90 110]  Measurements=None  LoadType=constant Z
  LG3-LMO 104km : powerlib/Elements/Distributed Parameters Line  Phases=3  Frequency=60  Resistance="[0.01273  0.3864]"  Inductance="[0.9337e-3  4.1264e-3]"  Capacitance=[12.74e-9 7.751e-9]  Length=104  x1=[-0.0006 -2.13713890637215e-09 0 0;-0.00056 -2.17493465222374e-09 0 0;-0.00052 -2.21223583669126e-09 0 0;-0.00048 -2.24903397780702e-09 0 0;-0.00044 -2.28532070799107e-09 0 0;-0.0004 -2.32108777595389e-09 0 0;-0.00036 -2.35632704857267e-09 584364.060408613 -381608.997671347;-0.00032 -2.3910305127407e-09 590051.873876247 -372753.99553941;-0.00028 -2.4251902771895e-09 595605.514636152 -363814.232363381;-0.00024 -2.45879857428322e-09 601023.719838313 -354791.740968313;-0.0002 -2.49184776178493e-09 606305.25742959 -345688.572990943;-0.00016 -2.52433032459438e-09 611448.926433881 -336506.798413165;-0.00012 -2.55623887645692e-09 616453.557225212 -327248.50509134;-8e-05 -2.58756616164302e-09 621318.011793699 -317915.798281528;-4e-05 -2.61830505659818e-09 626041.184004323 -308510.800160775]  x2=[-0.0006 2.19841025869437e-08 0 0;-0.00056 2.20831106292853e-08 0 0;-0.00052 2.21770971627064e-08 0 0;-0.00048 2.22660408154798e-08 0 0;-0.00044 2.2349921362586e-08 0 0;-0.0004 2.24287197303118e-08 0 0;-0.00036 2.2502418000588e-08 536183.908919966 -449688.611003349;-0.00032 2.25709994150635e-08 542903.776837676 -441552.382769491;-0.00028 2.2634448378916e-08 549500.193118335 -433315.749331577;-0.00024 2.26927504643982e-08 555971.657793768 -424980.583629021;-0.0002 2.27458924141188e-08 562316.699308713 -416548.781006624;-0.00016 2.27938621440567e-08 568533.874855448 -408022.25878359;-0.00012 2.28366487463089e-08 574621.770701868 -399402.955817543;-8e-05 2.28742424915711e-08 580579.002512958 -390692.832063647;-4e-05 2.29066348313497e-08 586404.215665577 -381893.868128931]  x3=[-0.0006 -1.93696080442392e-11 0 0;-0.00056 -1.71790832076202e-11 0 0;-0.00052 -1.49846519956259e-11 0 0;-0.00048 -1.278681340299e-11 0 0;-0.00044 -1.0586067199255e-11 0 0;-0.0004 -8.38291381512918e-12 0 0;-0.00036 -6.177854228693e-12 149.635910882607 -301.997984807482;-0.00032 -3.97138985148077e-12 154.172611510177 -299.707516419794;-0.00028 -1.76402241446412e-12 158.674254615418 -297.348897127439;-0.00024 4.43746146037295e-13 163.139816563507 -294.922663260106;-0.0002 2.65141380249181e-12 167.568281924168 -292.429366522452;-0.00016 4.85847855031245e-12 171.958643702567 -289.869573868654;-0.00012 7.06443852200849e-12 176.309903568296 -287.243867373487;-8e-05 9.26879210130574e-12 180.621072082385 -284.552844099966;-4e-05 1.14710380372098e-11 184.891168922293 -281.797115963575]  x4=[-0.0006 4.69524252049218e-11 0 0;-0.00056 4.48565808756731e-11 0 0;-0.00052 4.27505365467601e-11 0 0;-0.00048 4.06347711145012e-11 0 0;-0.00044 3.85097656857102e-11 0 0;-0.0004 3.63760034682964e-11 0 0;-0.00036 3.42339696613872e-11 3766.92032708438 -3037.04304680636;-0.00032 3.20841513449981e-11 3812.28758047003 -2979.89627382056;-0.00028 2.99270373692752e-11 3856.78795253564 -2922.07189811962;-0.00024 2.77631182433342e-11 3900.41132428037 -2863.58306846792;-0.0002 2.55928860237236e-11 3943.14777612568 -2804.44308472094;-0.00016 2.34168342025349e-11 3984.98759017095 -2744.66539480099;-0.00012 2.12354575951868e-11 4025.92125240329 -2684.26359163924;-8e-05 1.90492522279082e-11 4065.9394548609 -2623.25141008486;-4e-05 1.68587152249468e-11 4105.03309774964 -2561.64272378178]  x5=0.000588163229675572  V1=ones(3,3)  V2=ones(3,3)  I1=ones(3,3)  I2=ones(3,3)  nHarmo=1  Measurements=None
      settings: AttributesFormatString=\n  SourceProductName=Simscape Power Systems
  LG31-200 MVA : powerlib/Machines/Synchronous Machine pu Standard  PresetModel=No  MechanicalLoad=Mechanical power Pm  ShowDetailedParameters=on  RotorType=Salient-pole  Units=per unit standard parameters  MeasurementBus=off  NominalParameters="[200E6  13800   60 ]"  Reactances1=[ 31 32 33 34 35 36 37 ]  Reactances2=[ 1.305, 0.296, 0.252, 0.474, 0.243, 0.18 ]  dAxisTimeConstants=Short-circuit  qAxisTimeConstants=Open-circuit  TimeConstants1=[]  TimeConstants2=[]  TimeConstants3=[]  TimeConstants4=[]  TimeConstants5=[ 1.01, 0.053, 0.1 ]  TimeConstants6=[]  TimeConstants7=[]  TimeConstants8=[]  StatorResistance=2.8544e-3  Mechanical="[ 3.2  0  32]"  PolePairs=32  InitialConditions=[0 -66.4966 0.901556 0.901556 0.901556 -2.39998 -122.4 117.6 1.43992]  SetSaturation=off  Saturation=[0.6404,0.7127,0.8441,0.9214,0.9956,1.082,1.19,1.316,1.457;0.7,0.7698,0.8872,0.9466,0.9969,1.046,1.1,1.151,1.201]  LoadFlowParameters=[1 180000000 0 0 0]  TsPowergui=0  TsBlock=-1  IterativeModel=Trapezoidal non iterative  IterativeDiscreteModel=Trapezoidal non iterative  BusType=PV  Pref=180000000  Qref=0  Qmin=-Inf  Qmax=Inf  PLF=0  QLF=0
      settings: AttributesFormatString=\n\n  SourceProductName=Simscape Power Systems
  LG3_2200 MVA : powerlib/Machines/Synchronous Machine pu Standard  PresetModel=No  MechanicalLoad=Mechanical power Pm  ShowDetailedParameters=on  RotorType=Salient-pole  Units=per unit standard parameters  MeasurementBus=off  NominalParameters="[2200E6  13800   60 ]"  Reactances1=[ 31 32 33 34 35 36 37 ]  Reactances2=[ 1.305, 0.296, 0.252, 0.474, 0.243, 0.18 ]  dAxisTimeConstants=Short-circuit  qAxisTimeConstants=Open-circuit  TimeConstants1=[]  TimeConstants2=[]  TimeConstants3=[]  TimeConstants4=[]  TimeConstants5=[ 1.01, 0.053, 0.1 ]  TimeConstants6=[]  TimeConstants7=[]  TimeConstants8=[]  StatorResistance=2.8544e-3  Mechanical="[ 3.2  0  32]"  PolePairs=32  InitialConditions=[0 -68.8811 0.819571 0.819571 0.819571 -2.93694 -122.937 117.063 1.37344]  SetSaturation=off  Saturation=[0.6404,0.7127,0.8441,0.9214,0.9956,1.082,1.19,1.316,1.457;0.7,0.7698,0.8872,0.9466,0.9969,1.046,1.1,1.151,1.201]  LoadFlowParameters=[1 1800000000 0 0 0]  TsPowergui=0  TsBlock=-1  IterativeModel=Trapezoidal non iterative  IterativeDiscreteModel=Trapezoidal non iterative  BusType=PV  Pref=1800000000  Qref=0  Qmin=-Inf  Qmax=Inf  PLF=0  QLF=0
      settings: AttributesFormatString=\n\n  SourceProductName=Simscape Power Systems
  LG4 660 Mvar : powerlib/Elements/Three-Phase Series RLC Load  LConnTagsString=A|B|C  Configuration=Y (grounded)  NominalVoltage=735e3  Vabc=[1e3 1e3 1e3]  Vabcp=[1e3 1e3 1e3]  NominalFrequency=60  UnbalancedPower=off  ActivePower=2200000  InductivePower=660e6  CapacitivePower=0  Pabc=[10e3 9e3 11e3]  QLabc=[100 90 110]  QCabc=[100 90 110]  Pabcp=[10e3 9e3 11e3]  QLabcp=[100 90 110]  QCabcp=[100 90 110]  Measurements=None  LoadType=constant Z
  LG4-2700 MVA : powerlib/Machines/Synchronous Machine pu Standard  PresetModel=No  MechanicalLoad=Mechanical power Pm  ShowDetailedParameters=on  RotorType=Salient-pole  Units=per unit standard parameters  MeasurementBus=off  NominalParameters="[2700E6  13800   60 ]"  Reactances1=[ 31 32 33 34 35 36 37 ]  Reactances2=[ 1.305, 0.296, 0.252, 0.474, 0.243, 0.18 ]  dAxisTimeConstants=Short-circuit  qAxisTimeConstants=Open-circuit  TimeConstants1=[]  TimeConstants2=[]  TimeConstants3=[]  TimeConstants4=[]  TimeConstants5=[ 1.01, 0.053, 0.1 ]  TimeConstants6=[]  TimeConstants7=[]  TimeConstants8=[]  StatorResistance=2.8544e-3  Mechanical="[ 3.7  0  32]"  PolePairs=32  InitialConditions=[0 -68.0365 0.926345 0.926345 0.926345 -0.237768 -120.238 119.762 1.37332]  SetSaturation=off  Saturation=[0.6404,0.7127,0.8441,0.9214,0.9956,1.082,1.19,1.316,1.457;0.7,0.7698,0.8872,0.9466,0.9969,1.046,1.1,1.151,1.201]  LoadFlowParameters=[1 2500000000 0 0 0]  TsPowergui=0  TsBlock=-1  IterativeModel=Trapezoidal non iterative  IterativeDiscreteModel=Trapezoidal non iterative  BusType=PV  Pref=2500000000  Qref=0  Qmin=-Inf  Qmax=Inf  PLF=0  QLF=0
      settings: AttributesFormatString=\n\n  SourceProductName=Simscape Power Systems
  LG4-LMO 3*118km : powerlib/Elements/Distributed Parameters Line  Phases=3  Frequency=60  Resistance="[0.01273  0.3864]/3"  Inductance="[0.9337e-3  4.1264e-3]/3"  Capacitance=[12.74e-9 7.751e-9]*3  Length=118  x1=[-0.00068 4.27921691246115e-09 0 0;-0.00064 4.29564418341667e-09 0 0;-0.0006 4.31109466192894e-09 0 0;-0.00056 4.32556483469238e-09 0 0;-0.00052 4.33905141131449e-09 0 0;-0.00048 4.35155132506406e-09 0 0;-0.00044 4.36306173356849e-09 549437.198048253 -430432.644453508;-0.0004 4.37358001946015e-09 555865.199907066 -422098.763036803;-0.00036 4.38310379097152e-09 562166.802812998 -413668.900001409;-0.00032 4.39163088247911e-09 568340.57383589 -405144.972225483;-0.00028 4.39915935499584e-09 574385.109113453 -396528.917976694;-0.00024 4.40568749661197e-09 580299.034170489 -387822.696471477;-0.0002 4.41121382288441e-09 586081.00423144 -379028.287429523;-0.00016 4.41573707717421e-09 591729.704526177 -370147.690623608;-0.00012 4.41925623093235e-09 597243.850588964 -361182.925424864;-8e-05 4.42177048393362e-09 602622.188550538 -352136.030343586;-4e-05 4.42327926445857e-09 607863.495423229 -343009.0625657]  x2=[-0.00068 2.17000488167145e-08 0 0;-0.00064 2.1809665763703e-08 0 0;-0.0006 2.19143233807753e-08 0 0;-0.00056 2.2013997869692e-08 0 0;-0.00052 2.21086665653337e-08 0 0;-0.00048 2.21983079408555e-08 0 0;-0.00044 2.22829016125816e-08 522379.958057831 -465652.474678326;-0.0004 2.23624283446405e-08 529342.117405222 -457722.583925014;-0.00036 2.24368700533393e-08 536183.908919966 -449688.611003349;-0.00032 2.25062098112752e-08 542903.776837676 -441552.382769491;-0.00028 2.25704318511854e-08 549500.193118335 -433315.749331577;-0.00024 2.26295215695317e-08 555971.657793768 -424980.583629021;-0.0002 2.26834655298218e-08 562316.699308713 -416548.781006624;-0.00016 2.27322514656642e-08 568533.874855448 -408022.25878359;-0.00012 2.2775868283558e-08 574621.770701868 -399402.955817543;-8e-05 2.28143060654148e-08 580579.002512958 -390692.832063647;-4e-05 2.28475560708145e-08 586404.215665577 -381893.868128931]  x3=[-0.00068 -1.60397167763962e-11 0 0;-0.00064 -1.1645058123512e-11 0 0;-0.0006 -7.24775148483331e-12 0 0;-0.00056 -2.8487967699689e-12 0 0;-0.00052 1.55080573671403e-12 0 0;-0.00048 5.95005560354601e-12 0 0;-0.00044 1.03479524790448e-11 3083.93080468851 -3354.30372257589;-0.0004 1.47434963193869e-11 3134.1591857689 -3307.42032911895;-0.00036 1.91356876158084e-11 3183.67488607828 -3259.78485680115;-0.00032 2.35235276218852e-11 3232.46664617341 -3211.4081375181;-0.00028 2.79060185806391e-11 3280.52337122881 -3162.30117171858;-0.00024 3.22821639514189e-11 3327.83413355961 -3112.47512590314;-0.0002 3.66509686365058e-11 3374.38817510647 -3061.94133008491;-0.00016 4.10114392073892e-11 3420.17490988179 -3010.71127521327;-0.00012 4.53625841306644e-11 3465.18392637693 -2958.79661056092;-8e-05 4.97034139934986e-11 3509.40498992969 -2906.2091410749;-4e-05 5.40329417286146e-11 3552.82804505156 -2852.96082469229]  x4=[-0.00068 1.1399236713621e-10 0 0;-0.00064 1.10277507422276e-10 0 0;-0.0006 1.06537571554147e-10 0 0;-0.00056 1.02773409960988e-10 0 0;-0.00052 9.8985878580683e-11 0 0;-0.00048 9.51758386652072e-11 0 0;-0.00044 9.13441565847804e-11 7982.9563568463 -7444.85433654424;-0.0004 8.74917036308646e-11 8094.30988981071 -7323.63290932817;-0.00036 8.36193558180395e-11 8203.82284650852 -7200.74615114483;-0.00032 7.97279936848041e-11 8311.47032463779 -7076.22200538331;-0.00028 7.58185020933496e-11 8417.22784609031 -6950.08878776051;-0.00024 7.189177002835e-11 8521.07136251771 -6822.37517988238;-0.0002 6.79486903948141e-11 8622.97726079987 -6693.11022272201;-0.00016 6.39901598150471e-11 8722.9223684143 -6562.32331001591;-0.00012 6.00170784247657e-11 8820.88395870544 -6430.04418158018;-8e-05 5.60303496684158e-11 8916.83975605243 -6296.3029165479;-4e-05 5.20308800937364e-11 9010.76794093444 -6161.12992652941]  x5=0.000667339049054976  V1=ones(3,3)  V2=ones(3,3)  I1=ones(3,3)  I2=ones(3,3)  nHarmo=1  Measurements=None
      settings: AttributesFormatString=\n  SourceProductName=Simscape Power Systems
  LMO 330 Mvar : powerlib/Elements/Three-Phase Series RLC Load  LConnTagsString=A|B|C  Configuration=Y (grounded)  NominalVoltage=735e3  Vabc=[1e3 1e3 1e3]  Vabcp=[1e3 1e3 1e3]  NominalFrequency=60  UnbalancedPower=off  ActivePower=1100000  InductivePower=330e6  CapacitivePower=0  Pabc=[10e3 9e3 11e3]  QLabc=[100 90 110]  QCabc=[100 90 110]  Pabcp=[10e3 9e3 11e3]  QLabcp=[100 90 110]  QCabcp=[100 90 110]  Measurements=None  LoadType=constant Z
  LMO-ALB 3*218km : powerlib/Elements/Distributed Parameters Line  Phases=3  Frequency=60  Resistance="[0.01273  0.3864]/3"  Inductance="[0.9337e-3  4.1264e-3]/3"  Capacitance=[12.74e-9 7.751e-9]*3  Length=218  x1=[-0.00124 1.96606546756293e-08 360485.057850272 -599802.473105303;-0.0012 1.98365833280088e-08 369488.501232122 -594298.569189645;-0.00116 2.00080013124029e-08 378407.926115126 -588659.526904367;-0.00112 2.01748696498403e-08 387241.304298982 -582886.628519054;-0.00108 2.03371503958999e-08 395986.627149667 -576981.186741015;-0.00104 2.04948066493397e-08 404641.906056181 -570944.544416786;-0.001 2.0647802560487e-08 413205.172882742 -564778.074226773;-0.00096 2.07961033393912e-08 421674.480416318 -558483.178373119;-0.00092 2.09396752637339e-08 430047.902809414 -552061.288260856;-0.00088 2.10784856864978e-08 438323.536017986 -545513.864172417;-0.00084 2.12125030433896e-08 446499.498234409 -538842.394935577;-0.0008 2.13416968600182e-08 454573.930315381 -532048.397584907;-0.00076 2.14660377588238e-08 462544.996204677 -525133.417016816;-0.00072 2.15854974657583e-08 470410.883350655 -518099.025638253;-0.00068 2.17000488167145e-08 478169.80311841 -510946.823009156;-0.00064 2.1809665763703e-08 485819.991196497 -503678.435478724;-0.0006 2.19143233807753e-08 493359.707998118 -496295.515815602;-0.00056 2.2013997869692e-08 500787.239056694 -488799.742832054;-0.00052 2.21086665653337e-08 508100.895415713 -481192.821002216;-0.00048 2.21983079408555e-08 515299.01401279 -473476.480074512;-0.00044 2.22829016125816e-08 522379.958057831 -465652.474678326;-0.0004 2.23624283446405e-08 529342.117405222 -457722.583925014;-0.00036 2.24368700533393e-08 536183.908919966 -449688.611003349;-0.00032 2.25062098112752e-08 542903.776837676 -441552.382769491;-0.00028 2.25704318511854e-08 549500.193118335 -433315.749331577;-0.00024 2.26295215695317e-08 555971.657793768 -424980.583629021;-0.0002 2.26834655298218e-08 562316.699308713 -416548.781006624;-0.00016 2.27322514656642e-08 568533.874855448 -408022.25878359;-0.00012 2.2775868283558e-08 574621.770701868 -399402.955817543;-8e-05 2.28143060654148e-08 580579.002512958 -390692.832063647;-4e-05 2.28475560708145e-08 586404.215665577 -381893.868128931]  x2=[-0.00124 6.25331406005923e-08 229568.549789652 -648285.32022273;-0.0012 6.30688724337386e-08 239317.952112735 -644749.996709917;-0.00116 6.35902629491762e-08 249012.935597298 -641068.062607939;-0.00112 6.40971935871983e-08 258651.295687703 -637240.35515686;-0.00108 6.45895490761493e-08 268230.840703982 -633267.744744345;-0.00104 6.5067217458637e-08 277749.392340208 -629151.134707744;-0.001 6.55300901169903e-08 287204.786159826 -624891.461128678;-0.00096 6.59780617979585e-08 296594.872087819 -620489.692620186;-0.00092 6.64110306366444e-08 305917.514899625 -615946.830106468;-0.00088 6.68288981796678e-08 315170.594706663 -611263.906595282;-0.00084 6.72315694075531e-08 324352.00743838 -606441.986943053;-0.0008 6.76189527563354e-08 333459.665320698 -601482.167612725;-0.00076 6.7990960138382e-08 342491.497350756 -596385.576424444;-0.00072 6.83475069624222e-08 351445.449767838 -591153.372299093;-0.00068 6.86885121527829e-08 360319.486520378 -585786.744994772;-0.00064 6.90138981678246e-08 369111.589728947 -580286.914836248;-0.0006 6.93235910175734e-08 377819.760145094 -574655.132437472;-0.00056 6.9617520280546e-08 386442.017605963 -568892.678417195;-0.00052 6.98956191197627e-08 394976.401484562 -563000.863107767;-0.00048 7.01578242979458e-08 403420.971135596 -556981.02625718;-0.00044 7.04040761918988e-08 411773.806336747 -550834.536724423;-0.0004 7.06343188060646e-08 420033.007725323 -544562.79216821;-0.00036 7.08484997852584e-08 428196.697230154 -538167.218729166;-0.00032 7.10465704265725e-08 436263.018498645 -531649.270705541;-0.00028 7.12284856904511e-08 444230.137318901 -525010.430222504;-0.00024 7.1394204210932e-08 452096.242036809 -518252.206895133;-0.0002 7.15436883050527e-08 459859.543967989 -511376.13748513;-0.00016 7.16769039814193e-08 467518.277804531 -504383.785551383;-0.00012 7.17938209479358e-08 475070.702016406 -497276.741094422;-8e-05 7.18944126186924e-08 482515.099247478 -490056.620194868;-4e-05 7.19786561200104e-08 489849.776706014 -482725.06464595]  x3=[-0.00124 -4.98488964294288e-11 928.3722485006 -2076.19536430968;-0.0012 -4.29083731926369e-11 959.573235131517 -2061.96123480642;-0.00116 -3.59580929618071e-11 990.556023083773 -2047.25823309996;-0.00112 -2.89996361707271e-11 1021.31356713857 -2032.0897025261;-0.00108 -2.20345851124641e-11 1051.83887329563 -2016.45909227787;-0.00104 -1.50645235795647e-11 1082.12500036358 -2000.36995662127;-0.001 -8.09103650391428e-12 1112.1650615383 -1983.82595408698;-0.00096 -1.11570959633694e-12 1141.95222596892 -1966.83084663853;-0.00092 5.85987101398111e-12 1171.47972031113 -1949.38849881677;-0.00088 1.2834119140164e-11 1200.74083026736 -1931.50287686119;-0.00084 1.98054488983311e-11 1229.72890211353 -1913.17804780799;-0.0008 2.67722750682136e-11 1258.43734421209 -1894.41817856526;-0.00076 3.37330134536199e-11 1286.85962851088 -1875.22753496549;-0.00072 4.0686081242668e-11 1314.98929202755 -1855.61048079554;-0.00068 4.76298973677033e-11 1342.8199383192 -1835.57147680437;-0.00064 5.45628828648199e-11 1370.34523893686 -1815.11507968866;-0.0006 6.14834612329034e-11 1397.55893486454 -1794.24594105671;-0.00056 6.83900587921132e-11 1424.45483794247 -1772.96880637069;-0.00052 7.52811050417245e-11 1451.02683227422 -1751.28851386753;-0.00048 8.21550330172459e-11 1477.26887561744 -1729.20999345879;-0.00044 8.9010279646734e-11 1503.17500075776 -1706.73826560961;-0.0004 9.58452861062224e-11 1528.73931686575 -1683.87844019711;-0.00036 1.02658498174185e-10 1553.95601083636 -1660.63571534846;-0.00032 1.09448366584952e-10 1578.81934861085 -1637.01537625885;-0.00028 1.16213347380999e-10 1603.32367648063 -1613.0227939897;-0.00024 1.22951902264034e-10 1627.46342237286 -1588.66342424731;-0.0002 1.29662498944786e-10 1651.23309711748 -1563.9428061423;-0.00016 1.36343611491439e-10 1674.62729569544 -1538.86656093004;-0.00012 1.42993720676617e-10 1697.64069846774 -1513.44039073244;-8e-05 1.49611314322838e-10 1720.26807238503 -1487.67007724135;-4e-05 1.56194887646375e-10 1742.50427217762 -1461.56148040381]  x4=[-0.00124 3.19285792017316e-10 3596.66425144795 -12576.1807510608;-0.0012 3.16121497851999e-10 3785.89243012056 -12520.5172289183;-0.00116 3.12885320384185e-10 3974.25972950272 -12462.0066491303;-0.00112 3.09577995492724e-10 4161.72331649494 -12400.6623164981;-0.00108 3.06200275234776e-10 4348.24056349416 -12336.4981801938;-0.00104 3.02752927674797e-10 4533.76905808688 -12269.5288305888;-0.001 2.99236736709895e-10 4718.26661269334 -12199.7694959356;-0.00096 2.95652501891573e-10 4901.69127416068 -12127.2360389054;-0.00092 2.9200103824392e-10 5084.00133330265 -12051.9449529808;-0.00088 2.8828317607828e-10 5265.155334384 -11973.9133587054;-0.00084 2.84499760804447e-10 5445.11208454707 -11893.1589997908;-0.0008 2.80651652738429e-10 5623.83066317876 -11809.700239082;-0.00076 2.76739726906816e-10 5801.2704312155 -11723.5560543813;-0.00072 2.72764872847805e-10 5977.3910403842 -11634.7460341335;-0.00068 2.68727994408933e-10 6152.15244237714 -11543.2903729712;-0.00064 2.64630009541544e-10 6325.51489795859 -11449.2098671233;-0.0006 2.60471850092057e-10 6497.43898600117 -11352.5259096854;-0.00056 2.56254461590072e-10 6667.88561244985 -11253.2604857556;-0.00052 2.51978803033367e-10 6836.81601921166 -11151.4361674353;-0.00048 2.47645846669824e-10 7004.19179296889 -11047.0761086965;-0.00044 2.43256577776356e-10 7169.97487391397 -10940.2040401165;-0.0004 2.38811994434856e-10 7334.12756440396 -10830.844263482;-0.00036 2.34313107305249e-10 7496.61253753263 -10719.0216462632;-0.00032 2.29760939395671e-10 7657.39284561829 -10604.761615959;-0.00028 2.25156525829848e-10 7816.4319286054 -10488.0901543149;-0.00024 2.20500913611719e-10 7973.69362237799 -10369.0337914152;-0.0002 2.15795161387353e-10 8129.14216698305 -10247.61959965;-0.00016 2.11040339204226e-10 8282.74221476208 -10123.8751875596;-0.00012 2.06237528267899e-10 8434.4588383888 -9997.82869355606;-8e-05 2.0138782069616e-10 8584.25753881134 -9869.50877952523;-4e-05 1.96492319270689e-10 8732.10425309704 -9738.94462430897]  x5=0.00123288061605072  V1=ones(3,3)  V2=ones(3,3)  I1=ones(3,3)  I2=ones(3,3)  nHarmo=1  Measurements=None
      settings: AttributesFormatString=\n  SourceProductName=Simscape Power Systems
  LMO7 : powerlib/Measurements/Three-Phase V-I Measurement  VoltageMeasurement=no  SetLabelV=on  LabelV=Vabc_LMO7  Vpu=on  VpuLL=off  CurrentMeasurement=no  SetLabelI=off  LabelI=A1  Ipu=off  Pbase=100e6  Vbase=735e3  OutputType=Magnitude  PhasorSimulation=off  PSBequivalent=0
  LVD 990 Mvar : powerlib/Elements/Three-Phase Series RLC Load  LConnTagsString=A|B|C  Configuration=Y (grounded)  NominalVoltage=735e3  Vabc=[1e3 1e3 1e3]  Vabcp=[1e3 1e3 1e3]  NominalFrequency=60  UnbalancedPower=off  ActivePower=3300000  InductivePower=990e6  CapacitivePower=0  Pabc=[10e3 9e3 11e3]  QLabc=[100 90 110]  QCabc=[100 90 110]  Pabcp=[10e3 9e3 11e3]  QLabcp=[100 90 110]  QCabcp=[100 90 110]  Measurements=None  LoadType=constant Z
  LVD-MTL 3*260km : powerlib/Elements/Distributed Parameters Line  Phases=3  Frequency=60  Resistance="[0.01273  0.3864]/3"  Inductance="[0.9337e-3  4.1264e-3]/3"  Capacitance=[12.74e-9 7.751e-9]*3  Length=260  x1=[-0.00148 1.93286383652742e-07 6591.54381119535 -685037.200657489;-0.00144 1.95446012591388e-07 16920.4901046044 -684859.984797968;-0.0014 1.97561198792226e-07 27245.5888244798 -684527.037683885;-0.00136 1.99631461280153e-07 37564.4921324123 -684038.435024542;-0.00132 2.01656329295334e-07 47874.8535987765 -683394.287923971;-0.00128 2.03635342400243e-07 58174.3287362874 -682594.742855667;-0.00124 2.05568050584367e-07 68460.5755331176 -681639.981629284;-0.0012 2.07454014366531e-07 78731.2549854506 -680530.221349291;-0.00116 2.09292804894836e-07 88984.0316293492 -679265.714365607;-0.00112 2.11084004044171e-07 99216.574071821 -677846.748216213;-0.00108 2.12827204511298e-07 109426.555520956 -676273.645561777;-0.00104 2.14522009907463e-07 119611.65431502 -674546.764112276;-0.001 2.16168034848534e-07 129769.55445038 -672666.496545659;-0.00096 2.17764905042634e-07 139897.946108143 -670633.270418556;-0.00092 2.19312257375252e-07 149994.526179389 -668447.548069055;-0.00088 2.20809739991811e-07 160056.99878888 -666109.826511569;-0.00084 2.22257012377678e-07 170083.075817119 -663620.637323821;-0.0008 2.23653745435593e-07 180070.477420651 -660980.546525966;-0.00076 2.24999621560504e-07 190016.932550479 -658190.154451885;-0.00072 2.26294334711786e-07 199920.179468482 -655250.095612672;-0.00068 2.27537590482834e-07 209777.966261712 -652161.038552352;-0.00064 2.28729106168007e-07 219588.051354461 -648923.685695863;-0.0006 2.29868610826913e-07 229348.20401798 -645538.773189326;-0.00056 2.30955845346019e-07 239056.20487772 -642007.070732655;-0.00052 2.31990562497572e-07 248709.846418003 -638329.381404533;-0.00048 2.32972526995815e-07 258306.933483993 -634506.541479797;-0.00044 2.33901515550488e-07 267845.283780853 -630539.420239281;-0.0004 2.34777316917606e-07 277322.728369981 -626428.919772142;-0.00036 2.3559973194749e-07 286737.112162207 -622175.97477074;-0.00032 2.36368573630054e-07 296086.294407842 -617781.552318092;-0.00028 2.37083667137331e-07 305368.149183469 -613246.651667968;-0.00024 2.37744849863224e-07 314580.565875354 -608572.304017669;-0.0002 2.38351971460482e-07 323721.449659386 -603759.572273541;-0.00016 2.38904893874889e-07 332788.721977421 -598809.550809278;-0.00012 2.39403491376658e-07 341780.321009925 -593723.365217075;-8e-05 2.39847650589015e-07 350694.20214482 -588502.172051673;-4e-05 2.40237270513986e-07 359528.338442406 -583147.158567374]  x2=[-0.00148 2.95745357842407e-07 -242091.558410747 -615922.116309054;-0.00144 2.98818754458776e-07 -232776.518363146 -619502.655284383;-0.0014 3.01824202267284e-07 -223408.546942649 -622942.324698263;-0.00136 3.04761017855018e-07 -213989.774345171 -626240.342399533;-0.00132 3.07628533415438e-07 -204522.342318376 -629395.958447407;-0.00128 3.10426096900235e-07 -195008.403674663 -632408.455282011;-0.00124 3.13153072167598e-07 -185450.121801635 -635277.147887541;-0.0012 3.15808839126867e-07 -175849.670170163 -638001.383948039;-0.00116 3.18392793879538e-07 -166209.231840158 -640580.543995716;-0.00112 3.20904348856583e-07 -156530.99896416 -643014.041551821;-0.00108 3.2334293295206e-07 -146817.172288863 -645301.323259993;-0.00104 3.25707991652974e-07 -137069.960654684 -647441.869012097;-0.001 3.27998987165372e-07 -127291.580493494 -649435.192066489;-0.00096 3.30215398536632e-07 -117484.255324616 -651280.839158696;-0.00092 3.3235672177392e-07 -107650.215249218 -652978.390604485;-0.00088 3.344224699588e-07 -97791.6964432079 -654527.460395296;-0.00084 3.36412173357947e-07 -87910.9406487465 -655927.696286017;-0.0008 3.38325379529968e-07 -78010.1946644932 -657178.779875083;-0.00076 3.40161653428278e-07 -68091.7098347044 -658280.426676874;-0.00072 3.41920577500027e-07 -58157.7415372972 -659232.386186407;-0.00068 3.4360175178105e-07 -48210.5486709954 -660034.441936299;-0.00064 3.45204793986813e-07 -38252.3931416758 -660686.411545989;-0.0006 3.46729339599343e-07 -28285.5393480304 -661188.146763211;-0.00056 3.48175041950115e-07 -18312.2536666614 -661539.533497702;-0.00052 3.49541572298881e-07 -8334.80393672679 -661740.49184715;-0.00048 3.50828619908424e-07 1644.54105574682 -661790.976115359;-0.00044 3.52035892115218e-07 11623.5120937662 -661690.974822642;-0.0004 3.53163114395972e-07 21599.8400453724 -661440.51070843;-0.00036 3.54210030430062e-07 31571.2563796214 -661039.640726103;-0.00032 3.5517640215781e-07 41535.4936824286 -660488.456030038;-0.00028 3.56062009834617e-07 51490.2861721592 -659787.081954881;-0.00024 3.56866652080936e-07 61433.3702148476 -658935.67798705;-0.0002 3.57590145928059e-07 71362.484838928 -657934.437728463;-0.00016 3.58232326859724e-07 81275.3722493598 -656783.588852522;-0.00012 3.58793048849525e-07 91169.7783410311 -655483.393052336;-8e-05 3.59272184394117e-07 101043.453211322 -654034.145981219;-4e-05 3.59669624542209e-07 110894.151671715 -652436.177185455]  x3=[-0.00148 2.96282615116099e-10 785.9314472952 795.183399412992;-0.00144 3.19660518987467e-10 773.850798416553 806.943725754861;-0.0014 3.42965734813451e-10 761.59418253975 818.520560052279;-0.00136 3.66192963188949e-10 749.164386713547 829.911269832963;-0.00132 3.89336922442532e-10 736.564237366323 841.113264947736;-0.00128 4.1239234983745e-10 723.796599663382 852.123998159513;-0.00124 4.35354002768335e-10 710.864376855433 862.940965722512;-0.0012 4.58216659953324e-10 697.77050961842 873.561707951592;-0.00116 4.80975122621331e-10 684.517975384837 883.983809781559;-0.00112 5.03624215694207e-10 671.109787666683 894.204901316333;-0.00108 5.26158788963505e-10 657.548995370218 904.222658367843;-0.00104 5.48573718261592e-10 643.838682102667 914.034802984524;-0.001 5.70863906626845e-10 629.981965471034 923.639103969306;-0.00096 5.93024285462652e-10 615.981996373186 933.033377386971;-0.00092 6.15049815689968e-10 601.841958281365 942.215487060755;-0.00088 6.3693548889316e-10 587.565066518295 951.183345058101;-0.00084 6.58676328458875e-10 573.154567526044 959.934912165437;-0.0008 6.80267390707682e-10 558.613738127813 968.468198351873;-0.00076 7.01703766018217e-10 543.94588478281 976.781263221717;-0.00072 7.22980579943596e-10 529.154342834398 984.872216455708;-0.00068 7.44092994319815e-10 514.242475751657 992.739218240853;-0.00064 7.6503620836591e-10 499.213674364569 1000.38047968879;-0.0006 7.85805459775613e-10 484.071356092966 1007.79426324256;-0.00056 8.06396025800262e-10 468.818964169441 1014.97888307171;-0.00052 8.26803224322706e-10 453.459966856386 1021.93270545566;-0.00048 8.47022414921988e-10 437.997856657341 1028.65414915516;-0.00044 8.67048999928526e-10 422.436149522824 1035.14168577188;-0.0004 8.86878425469592e-10 406.77838405084 1041.39384009593;-0.00036 9.0650618250482e-10 391.02812068223 1047.40919044135;-0.00032 9.25927807851523e-10 375.18894089106 1053.18636896933;-0.00028 9.45138885199582e-10 359.264446370223 1058.7240619993;-0.00024 9.64135046115678e-10 343.258258212445 1064.02101030762;-0.0002 9.82911971036632e-10 327.174016086884 1069.07600941392;-0.00016 1.00146539025165e-09 311.015377411493 1073.887909855;-0.00012 1.01979108487319e-09 294.786016521361 1078.4556174462;-8e-05 1.03788488779633e-09 278.489623833198 1082.77809353019;-4e-05 1.05574268464633e-09 262.129905006168 1086.85435521319]  x4=[-0.00148 1.12840191469459e-09 -5816.93364762728 -14636.4207950644;-0.00144 1.13244701958605e-09 -5595.56829461436 -14722.4716350549;-0.0014 1.13623461579106e-09 -5372.93055762537 -14805.1747119568;-0.00136 1.1397638420429e-09 -5149.07106256176 -14884.5112198035;-0.00132 1.14303389582597e-09 -4924.04071314222 -14960.4631181575;-0.00128 1.14604403355824e-09 -4697.89067932763 -15033.0131362119;-0.00124 1.14879357076033e-09 -4470.67238568544 -15102.1447767183;-0.0012 1.15128188221121e-09 -4242.43749969618 -15167.8423197378;-0.00116 1.15350840209031e-09 -4013.23792000472 -15230.0908262158;-0.00112 1.1554726241062e-09 -3783.12576461894 -15288.8761413785;-0.00108 1.15717410161175e-09 -3552.15335905857 -15344.1848979524;-0.00104 1.15861244770563e-09 -3320.37322445681 -15396.0045192031;-0.001 1.15978733532035e-09 -3087.8380656175 -15444.3232217956;-0.00096 1.1606984972966e-09 -2854.60075903044 -15489.1300184736;-0.00092 1.161345726444e-09 -2620.71434084781 -15530.414720558;-0.00088 1.16172887558823e-09 -2386.23199482415 -15568.1679402636;-0.00084 1.16184785760447e-09 -2151.20704022285 -15602.3810928337;-0.0008 1.16170264543724e-09 -1915.69291969183 -15633.0463984925;-0.00076 1.16129327210654e-09 -1679.7431871111 -15660.1568842139;-0.00072 1.16061983070033e-09 -1443.41149541511 -15683.7063853073;-0.00068 1.15968247435337e-09 -1206.75158439251 -15703.6895468192;-0.00064 1.15848141621242e-09 -969.817268466202 -15720.101824751;-0.0006 1.15701692938774e-09 -732.662424456394 -15732.9394870922;-0.00056 1.15528934689101e-09 -495.340979329478 -15742.1996146692;-0.00052 1.15329906155959e-09 -257.9068979355 -15747.8801018087;-0.00048 1.1510465259672e-09 -20.4141707370256 -15749.979656817;-0.00044 1.148532252321e-09 217.08319846783 -15748.4978022734;-0.0004 1.14575681234515e-09 454.531204825399 -15743.4348751388;-0.00036 1.14272083715075e-09 691.875854706701 -15734.7920266792;-0.00032 1.13942501709239e-09 929.063177985127 -15722.5712222038;-0.00028 1.13587010161113e-09 1166.03924030878 -15706.7752406182;-0.00024 1.13205689906409e-09 1402.75015536468 -15687.4076737923;-0.0002 1.12798627654064e-09 1639.14209713205 -15664.4729257439;-0.00016 1.12365915966525e-09 1875.16131212189 -15637.9762116367;-0.00012 1.11907653238698e-09 2110.75413160006 -15607.9235565952;-8e-05 1.11423943675574e-09 2345.86698379107 -15574.321794334;-4e-05 1.10914897268538e-09 2580.44640605986 -15537.1785656039]  x5=0.00147040807418893  V1=ones(3,3)  V2=ones(3,3)  I1=ones(3,3)  I2=ones(3,3)  nHarmo=1  Measurements=None
      settings: AttributesFormatString=\n  SourceProductName=Simscape Power Systems
  LVD7 : powerlib/Measurements/Three-Phase V-I Measurement  VoltageMeasurement=no  SetLabelV=on  LabelV=Vabc_LVD7  Vpu=on  VpuLL=off  CurrentMeasurement=no  SetLabelI=off  LabelI=A1  Ipu=off  Pbase=100e6  Vbase=735e3  OutputType=Magnitude  PhasorSimulation=off  PSBequivalent=0
  Load Flow Bus1 : powerlib/Measurements/Load Flow Bus  LConnTagsString=a  Phases=single  Connectors=on one side  ID=LG31_13.8  Vbase=13.8e3  Vref=1  Vangle=0  VLF=1  VLFb=1  VLFc=1  angleLF=0.9665  angleLFb=0  angleLFc=0
      settings: AttributesFormatString=%<ID>\n%<Vbase>V\n%<VLF>pu\n%<angleLF>deg.  SourceProductName=Simscape Power Systems
  Load Flow Bus10 : powerlib/Measurements/Load Flow Bus  LConnTagsString=a  Phases=single  Connectors=on one side  ID=LVD7  Vbase=735e3  Vref=1  Vangle=0  VLF=1.045  VLFb=1  VLFc=1  angleLF=-9.599  angleLFb=0  angleLFc=0
      settings: AttributesFormatString=%<ID>\n%<Vbase>V\n%<VLF>pu\n%<angleLF>deg.  SourceProductName=Simscape Power Systems
  Load Flow Bus11 : powerlib/Measurements/Load Flow Bus  LConnTagsString=a  Phases=single  Connectors=on one side  ID=CHM7  Vbase=735e3  Vref=1  Vangle=0  VLF=1.045  VLFb=1  VLFc=1  angleLF=-1.818  angleLFb=0  angleLFc=0
      settings: AttributesFormatString=%<ID>\n%<Vbase>V\n%<VLF>pu\n%<angleLF>deg.  SourceProductName=Simscape Power Systems
  Load Flow Bus12 : powerlib/Measurements/Load Flow Bus  LConnTagsString=a  Phases=single  Connectors=on one side  ID=LG47  Vbase=735e3  Vref=1  Vangle=0  VLF=1.006  VLFb=1  VLFc=1  angleLF=22.05  angleLFb=0  angleLFc=0
      settings: AttributesFormatString=%<ID>\n%<Vbase>V\n%<VLF>pu\n%<angleLF>deg.  SourceProductName=Simscape Power Systems
  Load Flow Bus2 : powerlib/Measurements/Load Flow Bus  LConnTagsString=a  Phases=single  Connectors=on one side  ID=LG3_13.8  Vbase=13.8e3  Vref=1  Vangle=0  VLF=1  VLFb=1  VLFc=1  angleLF=0.4  angleLFb=0  angleLFc=0
      settings: AttributesFormatString=%<ID>\n%<Vbase>V\n%<VLF>pu\n%<angleLF>deg.  SourceProductName=Simscape Power Systems
  Load Flow Bus3 : powerlib/Measurements/Load Flow Bus  LConnTagsString=a  Phases=single  Connectors=on one side  ID=LG4_13.8  Vbase=13.8e3  Vref=1  Vangle=0  VLF=1  VLFb=1  VLFc=1  angleLF=-1.961  angleLFb=0  angleLFc=0
      settings: AttributesFormatString=%<ID>\n%<Vbase>V\n%<VLF>pu\n%<angleLF>deg.  SourceProductName=Simscape Power Systems
  Load Flow Bus4 : powerlib/Measurements/Load Flow Bus  LConnTagsString=a  Phases=single  Connectors=on one side  ID=LG2_13.8  Vbase=13.8e3  Vref=1  Vangle=0  VLF=1  VLFb=1  VLFc=1  angleLF=0  angleLFb=0  angleLFc=0
      settings: AttributesFormatString=%<ID>\n%<Vbase>V\n%<VLF>pu\n%<angleLF>deg.  SourceProductName=Simscape Power Systems
  Load Flow Bus5 : powerlib/Measurements/Load Flow Bus  LConnTagsString=a  Phases=single  Connectors=on one side  ID=LG27  Vbase=735e3  Vref=1  Vangle=0  VLF=1.003  VLFb=1  VLFc=1  angleLF=24.11  angleLFb=0  angleLFc=0
      settings: AttributesFormatString=%<ID>\n%<Vbase>V\n%<VLF>pu\n%<angleLF>deg.  SourceProductName=Simscape Power Systems
  Load Flow Bus6 : powerlib/Measurements/Load Flow Bus  LConnTagsString=a  Phases=single  Connectors=on one side  ID=LG37  Vbase=735e3  Vref=1  Vangle=0  VLF=0.9957  VLFb=1  VLFc=1  angleLF=25.11  angleLFb=0  angleLFc=0
      settings: AttributesFormatString=%<ID>\n%<Vbase>V\n%<VLF>pu\n%<angleLF>deg.  SourceProductName=Simscape Power Systems
  Load Flow Bus7 : powerlib/Measurements/Load Flow Bus  LConnTagsString=a  Phases=single  Connectors=on one side  ID=LMO7  Vbase=735e3  Vref=1  Vangle=0  VLF=1.019  VLFb=1  VLFc=1  angleLF=18.66  angleLFb=0  angleLFc=0
      settings: AttributesFormatString=%<ID>\n%<Vbase>V\n%<VLF>pu\n%<angleLF>deg.  SourceProductName=Simscape Power Systems
  Load Flow Bus8 : powerlib/Measurements/Load Flow Bus  LConnTagsString=a  Phases=single  Connectors=on one side  ID=NEM_ALB7  Vbase=735e3  Vref=1  Vangle=0  VLF=1.032  VLFb=1  VLFc=1  angleLF=10.49  angleLFb=0  angleLFc=0
      settings: AttributesFormatString=%<ID>\n%<Vbase>V\n%<VLF>pu\n%<angleLF>deg.  SourceProductName=Simscape Power Systems
  Load Flow Bus9 : powerlib/Measurements/Load Flow Bus  LConnTagsString=a  Phases=single  Connectors=on one side  ID=ABI_CHB7  Vbase=735e3  Vref=1  Vangle=0  VLF=1.047  VLFb=1  VLFc=1  angleLF=2.127  angleLFb=0  angleLFc=0
      settings: AttributesFormatString=%<ID>\n%<Vbase>V\n%<VLF>pu\n%<angleLF>deg.  SourceProductName=Simscape Power Systems
  NEM-ABI 6*236 : powerlib/Elements/Distributed Parameters Line  Phases=3  Frequency=60  Resistance="[0.01273  0.3864]/6"  Inductance="[0.9337e-3  4.1264e-3]/6"  Capacitance=[12.74e-9 7.751e-9]*6  Length=236  x1=[-0.00136 5.887073204798e-08 0 0;-0.00132 5.94377824370773e-08 0 0;-0.00128 5.99913171870179e-08 0 0;-0.00124 6.05312104287733e-08 0 0;-0.0012 6.10573393952762e-08 0 0;-0.00116 6.15695844493366e-08 0 0;-0.00112 6.20678291108467e-08 0 0;-0.00108 6.25519600832672e-08 0 0;-0.00104 6.30218672793899e-08 0 0;-0.001 6.34774438463707e-08 0 0;-0.00096 6.3918586190027e-08 0 0;-0.00092 6.43451939983941e-08 0 0;-0.00088 6.47571702645352e-08 0 0;-0.00084 6.51544213086003e-08 352358.048754719 -596372.974308211;-0.0008 6.55368567991276e-08 361310.690854675 -590991.996642238;-0.00076 6.59043897735845e-08 370181.174019342 -585476.632492727;-0.00072 6.62569366581422e-08 378967.481177344 -579828.136005922;-0.00068 6.65944172866793e-08 387667.614398202 -574047.791601214;-0.00064 6.69167549190112e-08 396279.595346648 -568136.913679073;-0.0006 6.72238762583401e-08 404801.465732483 -562096.846322165;-0.00056 6.75157114679218e-08 413231.28775587 -555928.962989721;-0.00052 6.77921941869464e-08 421567.144547975 -549634.66620522;-0.00048 6.80532615456279e-08 429807.140606851 -543215.387237472;-0.00044 6.82988541795003e-08 437949.402228451 -536672.585775155;-0.0004 6.85289162429164e-08 445992.0779327 -530007.749594901;-0.00036 6.87433954217472e-08 453933.338884498 -523222.394222981;-0.00032 6.89422429452768e-08 461771.379309589 -516318.062590693;-0.00028 6.91254135972932e-08 469504.416905171 -509296.324683508;-0.00024 6.92928657263698e-08 477130.693245183 -502158.777184075;-0.0002 6.94445612553364e-08 484648.474180151 -494907.043109144;-0.00016 6.9580465689938e-08 492056.05023152 -487542.771440505;-0.00012 6.97005481266781e-08 499351.736980378 -480067.636750031;-8e-05 6.98047812598461e-08 506533.875450472 -472483.338818888;-4e-05 6.98931413877263e-08 513600.832485451 -464791.602251019]  x2=[-0.00136 1.03630604361012e-07 0 0;-0.00132 1.04659626211625e-07 0 0;-0.00128 1.05664849365783e-07 0 0;-0.00124 1.06646045244411e-07 0 0;-0.0012 1.07602990732026e-07 0 0;-0.00116 1.08535468227477e-07 0 0;-0.00112 1.09443265693423e-07 0 0;-0.00108 1.1032617670455e-07 0 0;-0.00104 1.11184000494506e-07 0 0;-0.001 1.12016542001559e-07 0 0;-0.00096 1.12823611912951e-07 0 0;-0.00092 1.13605026707943e-07 0 0;-0.00088 1.1436060869955e-07 0 0;-0.00084 1.15090186074943e-07 196182.30408902 -655022.816531851;-0.0008 1.15793592934517e-07 206037.09013961 -651990.149855995;-0.00076 1.1647066932962e-07 215845.025132691 -648809.226242585;-0.00072 1.17121261298918e-07 225603.878828425 -645480.76900622;-0.00068 1.17745220903406e-07 235311.432147638 -642005.535009372;-0.00064 1.18342406260053e-07 244965.477676421 -638384.314490283;-0.0006 1.18912681574058e-07 254563.820168072 -634617.930883271;-0.00056 1.19455917169732e-07 264104.277042281 -630707.240631487;-0.00052 1.19971989519986e-07 273584.67888143 -626653.132992172;-0.00048 1.20460781274417e-07 283002.869923895 -622456.529834441;-0.00044 1.20922181285996e-07 292356.708554252 -618118.385429662;-0.0004 1.21356084636339e-07 301644.06779026 -613639.686234462;-0.00036 1.21762392659566e-07 310862.835766521 -609021.450666416;-0.00032 1.22141012964737e-07 320010.916214695 -604264.728872466;-0.00028 1.22491859456858e-07 329086.228940178 -599370.602490127;-0.00024 1.22814852356464e-07 338086.71029512 -594340.184401534;-0.0002 1.23109918217754e-07 347010.313647676 -589174.618480379;-0.00016 1.23376989945296e-07 355855.009847397 -583875.079331807;-0.00012 1.23616006809282e-07 364618.787686643 -578442.77202532;-8e-05 1.2382691445934e-07 373299.654357907 -572878.931820752;-4e-05 1.24009664936886e-07 381895.635906969 -567184.823887385]  x3=[-0.00136 5.32938338296341e-11 0 0;-0.00132 7.1150255221054e-11 0 0;-0.00128 8.89904976580101e-11 0 0;-0.00124 1.0681050442322e-10 0 0;-0.0012 1.24606223400819e-10 0 0;-0.00116 1.42373607997774e-10 0 0;-0.00112 1.60108618064049e-10 0 0;-0.00108 1.77807220811294e-10 0 0;-0.00104 1.9546539172987e-10 0 0;-0.001 2.13079115503989e-10 0 0;-0.00096 2.30644386924759e-10 0 0;-0.00092 2.48157211800934e-10 0 0;-0.00088 2.65613607867162e-10 0 0;-0.00084 2.83009605689516e-10 1033.96667826049 -3078.51753948798;-0.0008 3.00341249568106e-10 1080.26900983346 -3062.57757804577;-0.00076 3.17604598436577e-10 1126.32569754944 -3045.94121287285;-0.00072 3.3479572675827e-10 1172.12626851482 -3028.6122269352;-0.00068 3.51910725418853e-10 1217.66030807472 -3010.59456069479;-0.00064 3.68945702615224e-10 1262.91746218122 -2991.89231121353;-0.0006 3.85896784740473e-10 1307.88743974776 -2972.50973122169;-0.00056 4.02760117264704e-10 1352.56001498924 -2952.45122815079;-0.00052 4.19531865611525e-10 1396.9250297473 -2931.72136313148;-0.00048 4.36208216029994e-10 1440.97239580015 -2910.32484995627;-0.00044 4.52785376461837e-10 1484.69209715662 -2888.26655400776;-0.0004 4.69259577403728e-10 1528.07419233364 -2865.55149115221;-0.00036 4.85627072764439e-10 1571.10881661687 -2842.18482659904;-0.00032 5.01884140716673e-10 1613.78618430386 -2818.17187372626;-0.00028 5.18027084543373e-10 1656.09659092924 -2793.51809287227;-0.00024 5.34052233478323e-10 1698.03041547142 -2768.22909009424;-0.0002 5.4995594354085e-10 1739.57812254031 -2742.31061589332;-0.00016 5.65734598364434e-10 1780.73026454561 -2715.76856390701;-0.00012 5.81384610019038e-10 1821.47748384512 -2688.60896956907;-8e-05 5.9690241982697e-10 1861.81051487256 -2660.83800873702;-4e-05 6.12284499172101e-10 1901.72018624449 -2632.46199628787]  x4=[-0.00136 9.4976569106716e-10 0 0;-0.00132 9.4866287069979e-10 0 0;-0.00128 9.47344332576544e-10 0 0;-0.00124 9.45810376521619e-10 0 0;-0.0012 9.44061351343394e-10 0 0;-0.00116 9.42097654755112e-10 0 0;-0.00112 9.39919733284443e-10 0 0;-0.00108 9.37528082171948e-10 0 0;-0.00104 9.34923245258464e-10 0 0;-0.001 9.32105814861444e-10 0 0;-0.00096 9.29076431640262e-10 0 0;-0.00092 9.2583578445054e-10 0 0;-0.00088 9.223846101875e-10 0 0;-0.00084 9.18723693618411e-10 6756.67913073754 -26294.4191938105;-0.0008 9.14853867204128e-10 7152.40602451493 -26189.5466886012;-0.00076 9.10776010909807e-10 7546.50652284208 -26078.7189063239;-0.00072 9.06491052004802e-10 7938.89101066422 -25961.9610482606;-0.00068 9.01999964851818e-10 8329.47026313263 -25839.2996641414;-0.00064 8.97303770685343e-10 8718.15546589349 -25710.7626461072;-0.0006 8.92403537379432e-10 9104.85823528358 -25576.3792223674;-0.00056 8.87300379204881e-10 9489.49063842791 -25436.1799505538;-0.00052 8.81995456575852e-10 9871.96521323495 -25290.1967107716;-0.00048 8.76489975786002e-10 10252.1949882847 -25138.4626983508;-0.00044 8.70785188734186e-10 10630.0935026053 -24981.0124162973;-0.0004 8.64882392639784e-10 11005.5748253334 -24817.8816674474;-0.00036 8.58782929747723e-10 11378.5535752543 -24649.1075463266;-0.00032 8.52488187023267e-10 11748.9449402166 -24474.7284307146;-0.00028 8.45999595836626e-10 12116.6646964181 -24294.7839729186;-0.00024 8.39318631637482e-10 12481.6292275573 -24109.3150907564;-0.0002 8.32446813619479e-10 12843.7555438471 -23918.3639582524;-0.00016 8.25385704374775e-10 13202.9613008861 -23721.9739960475;-0.00012 8.18136909538719e-10 13559.1648183828 -23520.1898615255;-8e-05 8.10702077424746e-10 13912.285098729 -23313.0574386585;-4e-05 8.03082898649563e-10 14262.2418454182 -23100.6238275732]  x5=0.00133467809810995  V1=ones(3,3)  V2=ones(3,3)  I1=ones(3,3)  I2=ones(3,3)  nHarmo=1  Measurements=None
      settings: AttributesFormatString=\n  SourceProductName=Simscape Power Systems
  NEM-ALB 1980 Mvar : powerlib/Elements/Three-Phase Series RLC Load  LConnTagsString=A|B|C  Configuration=Y (grounded)  NominalVoltage=735e3  Vabc=[1e3 1e3 1e3]  Vabcp=[1e3 1e3 1e3]  NominalFrequency=60  UnbalancedPower=off  ActivePower=6600000  InductivePower=1980e6  CapacitivePower=0  Pabc=[10e3 9e3 11e3]  QLabc=[100 90 110]  QCabc=[100 90 110]  Pabcp=[10e3 9e3 11e3]  QLabcp=[100 90 110]  QCabcp=[100 90 110]  Measurements=None  LoadType=constant Z
  NEM-ALB7 : powerlib/Measurements/Three-Phase V-I Measurement  VoltageMeasurement=no  SetLabelV=on  LabelV=Vabc_NEM7  Vpu=on  VpuLL=off  CurrentMeasurement=no  SetLabelI=off  LabelI=A1  Ipu=off  Pbase=100e6  Vbase=735e3  OutputType=Magnitude  PhasorSimulation=off  PSBequivalent=0
  Regulators1 : Subsystem
  Regulators2 : Subsystem
  Regulators3 : Subsystem
  Regulators4 : Subsystem
  MTLa : PMIOPort  Port=1  Side=Right
  MTLb : PMIOPort  Port=2  Side=Right
  MTLc : PMIOPort  Port=3  Side=Right
  CHM7a : PMIOPort  Port=4  Side=Right
  CHM7b : PMIOPort  Port=5  Side=Right
  CHM7c : PMIOPort  Port=6  Side=Right
  wires:
  Regulators2/1(Pm) -> LG3_2200 MVA/1
  Regulators4/2(Vf) -> LG4-2700 MVA/2
  Regulators4/1(Pm) -> LG4-2700 MVA/1
  Regulators3/2(Vf) -> LG31-200 MVA/2
  Regulators3/1(Pm) -> LG31-200 MVA/1
  Regulators2/2(Vf) -> LG3_2200 MVA/2
  LG3_2200 MVA/1 -> Regulators2/1(m)
  Regulators1/1(Pm) -> LG2_5500 MVA/1
  Regulators1/2(Vf) -> LG2_5500 MVA/2
  LG2_5500 MVA/1 -> Regulators1/1(m)
  LG31-200 MVA/1 -> Regulators3/1(m)
  LG4-2700 MVA/1 -> Regulators4/1(m)
  connections:
  LG2-NENI 3*279km/RConn1 -- "Cs NEM "/LConn1
  LG2-NENI 3*279km/RConn2 -- "Cs NEM "/LConn2
  LG2-NENI 3*279km/RConn3 -- "Cs NEM "/LConn3
  CHB-CHM 3*195km/RConn1 -- "Cs  CHMN "/LConn1
  CHB-CHM 3*195km/RConn2 -- "Cs  CHMN "/LConn2
  CHB-CHM 3*195km/RConn3 -- "Cs  CHMN "/LConn3
  Load Flow Bus2/LConn1 -- 2200 MVA 13.8 kV/735 kV/LConn1 -- LG3_2200 MVA/RConn1 -- 110 MW/LConn1
  2200 MVA 13.8 kV/735 kV/LConn2 -- LG3_2200 MVA/RConn2 -- 110 MW/LConn2
  2200 MVA 13.8 kV/735 kV/LConn3 -- LG3_2200 MVA/RConn3 -- 110 MW/LConn3
  Load Flow Bus1/LConn1 -- 200 MVA 13.8 kV/735 kV/LConn1 -- LG31-200 MVA/RConn1 -- 10 MW/LConn1
  200 MVA 13.8 kV/735 kV/LConn2 -- LG31-200 MVA/RConn2 -- 10 MW/LConn2
  200 MVA 13.8 kV/735 kV/LConn3 -- LG31-200 MVA/RConn3 -- 10 MW/LConn3
  Load Flow Bus6/LConn1 -- 2200 MVA 13.8 kV/735 kV/RConn1 -- 200 MVA 13.8 kV/735 kV/RConn1 -- LG3-LMO 104km/LConn1 -- LG3 660 Mvar/LConn1 -- LG2-LG3 155km/RConn1
  2200 MVA 13.8 kV/735 kV/RConn2 -- LG3 660 Mvar/LConn2 -- LG2-LG3 155km/RConn2 -- 200 MVA 13.8 kV/735 kV/RConn2 -- LG3-LMO 104km/LConn2
  LG3-LMO 104km/RConn1 -- LMO7/RConn1 -- LG4-LMO 3*118km/RConn1 -- LMO 330 Mvar/LConn1
  LG3-LMO 104km/RConn2 -- LMO7/RConn2 -- LG4-LMO 3*118km/RConn2 -- LMO 330 Mvar/LConn2
  LG3-LMO 104km/RConn3 -- LMO7/RConn3 -- LG4-LMO 3*118km/RConn3 -- LMO 330 Mvar/LConn3
  LG4-LMO 3*118km/LConn1 -- LG4 660 Mvar/LConn1 -- 2700 MVA 13.8 kV/735 kV/RConn1 -- Load Flow Bus12/LConn1
  LG4-LMO 3*118km/LConn2 -- 2700 MVA 13.8 kV/735 kV/RConn2 -- LG4 660 Mvar/LConn2
  LG4 660 Mvar/LConn3 -- 2700 MVA 13.8 kV/735 kV/RConn3 -- LG4-LMO 3*118km/LConn3
  Load Flow Bus3/LConn1 -- LG4-2700 MVA/RConn1 -- 2700 MVA 13.8 kV/735 kV/LConn1 -- 135 MW/LConn1
  LG4-2700 MVA/RConn2 -- 2700 MVA 13.8 kV/735 kV/LConn2 -- 135 MW/LConn2
  LG4-2700 MVA/RConn3 -- 2700 MVA 13.8 kV/735 kV/LConn3 -- 135 MW/LConn3
  Load Flow Bus4/LConn1 -- 5500 MVA 13.8 kV/735 kV/LConn1 -- LG2_5500 MVA/RConn1 -- 275 MW/LConn1
  5500 MVA 13.8 kV/735 kV/LConn2 -- LG2_5500 MVA/RConn2 -- 275 MW/LConn2
  LG2_5500 MVA/RConn3 -- 5500 MVA 13.8 kV/735 kV/LConn3 -- 275 MW/LConn3
  5500 MVA 13.8 kV/735 kV/RConn1 -- LG2-NENI 3*279km/LConn1 -- LG2-LG3 155km/LConn1 -- LG2 660 Mvar/LConn1 -- Load Flow Bus5/LConn1
  LG2-LG3 155km/LConn2 -- 5500 MVA 13.8 kV/735 kV/RConn2 -- LG2-NENI 3*279km/LConn2 -- LG2 660 Mvar/LConn2
  LG2-LG3 155km/LConn3 -- 5500 MVA 13.8 kV/735 kV/RConn3 -- LG2-NENI 3*279km/LConn3 -- LG2 660 Mvar/LConn3
  "Cs NEM "/RConn1 -- NEM-ALB7/LConn1 -- Cs ALB/RConn1
  "Cs NEM "/RConn2 -- NEM-ALB7/LConn2 -- Cs ALB/RConn2
  "Cs NEM "/RConn3 -- NEM-ALB7/LConn3 -- Cs ALB/RConn3
  LMO7/LConn1 -- LMO-ALB 3*218km/LConn1
  LMO7/LConn2 -- LMO-ALB 3*218km/LConn2
  Load Flow Bus7/LConn1 -- LMO7/LConn3 -- LMO-ALB 3*218km/LConn3
  Cs ALB/LConn1 -- LMO-ALB 3*218km/RConn1
  Cs ALB/LConn2 -- LMO-ALB 3*218km/RConn2
  Cs ALB/LConn3 -- LMO-ALB 3*218km/RConn3
  200 MVA 13.8 kV/735 kV/RConn3 -- LG3-LMO 104km/LConn3 -- LG3 660 Mvar/LConn3 -- LG2-LG3 155km/RConn3 -- 2200 MVA 13.8 kV/735 kV/RConn3
  Load Flow Bus8/LConn1 -- NEM-ABI 6*236/LConn1 -- NEM-ALB7/RConn1 -- NEM-ALB 1980 Mvar/LConn1
  NEM-ALB 1980 Mvar/LConn2 -- NEM-ALB7/RConn2 -- NEM-ABI 6*236/LConn2
  NEM-ALB 1980 Mvar/LConn3 -- NEM-ALB7/RConn3 -- NEM-ABI 6*236/LConn3
  NEM-ABI 6*236/RConn1 -- "Cs ABI+CHB "/LConn1
  NEM-ABI 6*236/RConn2 -- "Cs ABI+CHB "/LConn2
  NEM-ABI 6*236/RConn3 -- "Cs ABI+CHB "/LConn3
  "Cs ABI+CHB "/RConn1 -- ABI-CHB7/LConn1
  "Cs ABI+CHB "/RConn2 -- ABI-CHB7/LConn2
  "Cs ABI+CHB "/RConn3 -- ABI-CHB7/LConn3
  Load Flow Bus9/LConn1 -- ABI+CHB 1320 Mvar/LConn1 -- CHB-CHM 3*195km/LConn1 -- ABI-CHB 3*271km/LConn1 -- ABI-CHB7/RConn1
  ABI-CHB 3*271km/LConn2 -- ABI-CHB7/RConn2 -- ABI+CHB 1320 Mvar/LConn2 -- CHB-CHM 3*195km/LConn2
  ABI-CHB 3*271km/LConn3 -- ABI-CHB7/RConn3 -- ABI+CHB 1320 Mvar/LConn3 -- CHB-CHM 3*195km/LConn3
  ABI-CHB 3*271km/RConn1 -- "Cs LVDN "/LConn1
  ABI-CHB 3*271km/RConn2 -- "Cs LVDN "/LConn2
  ABI-CHB 3*271km/RConn3 -- "Cs LVDN "/LConn3
  "Cs LVDN "/RConn1 -- LVD7/LConn1
  "Cs LVDN "/RConn2 -- LVD7/LConn2
  "Cs LVDN "/RConn3 -- LVD7/LConn3
  "Cs LVDS "/LConn1 -- LVD 990 Mvar/LConn1 -- Load Flow Bus10/LConn1 -- LVD7/RConn1
  "Cs LVDS "/LConn2 -- LVD7/RConn2 -- LVD 990 Mvar/LConn2
  "Cs LVDS "/LConn3 -- LVD7/RConn3 -- LVD 990 Mvar/LConn3
  "Cs LVDS "/RConn1 -- LVD-MTL 3*260km/LConn1
  "Cs LVDS "/RConn2 -- LVD-MTL 3*260km/LConn2
  "Cs LVDS "/RConn3 -- LVD-MTL 3*260km/LConn3
  MTLa/RConn1 -- LVD-MTL 3*260km/RConn1
  MTLb/RConn1 -- LVD-MTL 3*260km/RConn2
  MTLc/RConn1 -- LVD-MTL 3*260km/RConn3
  "Cs  CHMN "/RConn1 -- CHM7/LConn1
  "Cs  CHMN "/RConn2 -- CHM7/LConn2
  "Cs  CHMN "/RConn3 -- CHM7/LConn3
  CHM 1320Mvar/LConn2 -- CHM7/RConn2 -- CHM7b/RConn1
  Load Flow Bus11/LConn1 -- CHM 1320Mvar/LConn3 -- CHM7c/RConn1 -- CHM7/RConn3
  CHM7a/RConn1 -- CHM 1320Mvar/LConn1 -- CHM7/RConn1
